simulink library "xbsIndex_r4"  (Simulink 7.1)
(part 5 of 9)

      | nport = get_param(gcbh, 'ports');
      | nin = nport(1);
      | nout = nport(2);
      | 
      |   serialized_declarations = '{''Coefficient_Binary_Point''=>''Int'',''Coefficient_Buffer_Type''=>''Int'',''Coefficient_Reload''=>''Int'',''Coefficient_Sign''=>''Int'',''Coefficient_Structure''=>''Int'',''Coefficient_Width''=>''Int'',''Coefficients''=>''DoubleVector'',''Column_Wrap_Length''=>''Int'',''Data_Buffer_Type''=>''Int'',''Display_Block_Info''=>''Int'',''Enable_Port''=>''Int'',''Filter_Type''=>''Int'',''First_Column_Length''=>''Int'',''Hardware_Oversampling''=>''Int'',''Inter_Column_Pipe_Length''=>''Int'',''Multiple_Column_Support''=>''Int'',''Number_Channels''=>''Int'',''Rate_Change''=>''Int'',''Rst_Rfd_Port''=>''Int'',''Storage''=>''Int'',''Valid_Ports''=>''Int'',''Zero_Pack_Factor''=>''Int'',''enable_debug''=>''Int'',''u_coef_cols''=>''Int'',''u_coef_rows''=>''Int'',''u_coef_sets''=>''Int'',''u_coef_type''=>''Int'',''u_latency''=>''Int'',''block_type''=>''String'',''nin''=>''Double'',''nout''=>''Double''}';
      |   xlFir_compiler_v3_0_init();
      |   ptable_ = xlblockprep(get_param(tmp_gcb, 'MaskWSVariables'));
      |   try
      |     xlBlockMoveCallback(tmp_gcbh);
      |   catch 
      |      clear global xl_updateicon_recursion_guard;
      |   end;
      | catch
      |   global dbgsysgen;
      |   if(~isempty(dbgsysgen) && dbgsysgen)
      |     e = regexprep(lasterr, '\n', '\nError: ');
      |     disp(['Error: While running MaskInit code on block ' tmp_gcb ': ' e]);
      |     error(e);
      |   end
      | end
      settings: CopyFcn=xlBlockMoveCallback(gcbh);  DeleteFcn=xlDestroyGui(gcbh);  ModelCloseFcn=xlDestroyGui(gcbh);  PreSaveFcn=xlBlockPreSaveCallback(gcbh);  PostSaveFcn=xlBlockPostSaveCallback(gcbh);  DestroyFcn=xlDestroyGui(gcbh);  OpenFcn=xlOpenGui(gcbh, 'Fir_compiler_v3_0_gui.xml', @xlremovedenablement, -1)  CloseFcn=xlDestroyGui(gcbh);  MoveFcn=xlBlockMoveCallback(gcbh);
      mask Help: eval('');xlDoc('-book','sysgen','-topic','FIR_Compiler_v3_0');
      mask StyleString: edit,edit,popup(Single_Rate|Decimation|Interpolation|Interpolated),edit,edit,edit,edit,edit,edit,popup(Signed|Unsigned),edit,edit,edit,popup(Inferred|Non_Symmetric|Symmetric|Negative_Symmetric|Half_Band),edit,checkbox,edit,checkbox,edit,checkbox,edit,checkbox,edit,checkbox,edit,checkbox,edit,popup(Automatic|Custom),edit,popup(Distributed|Block),edit,popup(Distributed|Block),edit,popup(Disabled|Custom),edit,popup(1|2|3|4|5|6|7|8|9|10|11|12|13|14|15|16),edit,edit,edit,checkbox,edit,edit,edit,edit,edit,edit,edit,edit,edit,edit,edit,edit,edit,edit,edit
      mask Display:
      | fprintf('','COMMENT: begin icon graphics');
      | patch([0 90 90 0 0 ],[0 0 134 134 0 ],[0.77 0.82 0.91 ]);
      | plot([0 90 90 0 0 ],[0 0 134 134 0 ]);
      | patch([18.3 35.64 47.64 59.64 71.64 47.64 30.3 18.3 ],[80.32 80.32 92.32 80.32 92.32 92.32 92.32 80.32 ],[1 1 1 ]);
      | patch([30.3 47.64 35.64 18.3 30.3 ],[68.32 68.32 80.32 80.32 68.32 ],[0.931 0.946 0.973 ]);
      | patch([18.3 35.64 47.64 30.3 18.3 ],[56.32 56.32 68.32 68.32 56.32 ],[1 1 1 ]);
      | patch([30.3 71.64 59.64 47.64 35.64 18.3 30.3 ],[44.32 44.32 56.32 44.32 56.32 56.32 44.32 ],[0.931 0.946 0.973 ]);
      | fprintf('','COMMENT: end icon graphics');
      | fprintf('','COMMENT: begin icon text');
      | fprintf('','COMMENT: end icon text');
  "FIR Compiler v3_1 " : S-Function  LoadFcn=xlBlockLoadCallback(gcbh);  FunctionName=sysgen  Parameters=ptable_  EnableBusSupport=off  mask(Xilinx FIR Compiler v3_1 Block){infoedit=Implements a high-speed multi-channel FIR filter.<br><br>Hardware  notes: Implemented using DSP48s hence only Virtex 4, Virtex 5 and SpartanDSP devices are supported., Filter_Type_sgadvanced=, Filter_Type=Single_Rate, Rate_Change=1, Zero_Pack_Factor=1, Number_Channels=1, Hardware_Oversampling=1, Coefficients=[1 2 3], Coefficient_Sign_sgadvanced=, Coefficient_Sign=Signed, Coefficient_Width=16, Coefficient_Binary_Point=8, Coefficient_Structure_sgadvanced=, Coefficient_Structure=Inferred, Coefficient_Reload_sgadvanced=, Coefficient_Reload=off, Display_Block_Info_sgadvanced=, Display_Block_Info=off, Valid_Ports_sgadvanced=, Valid_Ports=off, Enable_Port_sgadvanced=, Enable_Port=off, Rst_Rfd_Port_sgadvanced=, Rst_Rfd_Port=off, Output_Rounding_Mode_sgadvanced=, Output_Rounding_Mode=Full_Precision, Output_Width=48, Allow_Rounding_Approximation_sgadvanced=, Allow_Rounding_Approximation=off, dbl_ovrd_sgadvanced=, dbl_ovrd=off, Storage_sgadvanced=, Storage=Automatic, Data_Buffer_Type_sgadvanced=, Data_Buffer_Type=Distributed, Coefficient_Buffer_Type_sgadvanced=, Coefficient_Buffer_Type=Distributed, Multiple_Column_Support_sgadvanced=, Multiple_Column_Support=Disabled, Inter_Column_Pipe_Length_sgadvanced=, Inter_Column_Pipe_Length=4, First_Column_Length=32, Column_Wrap_Length=32, xl_use_area_sgadvanced=, xl_use_area=off, xl_area=[0,0,0,0,0,0,0], u_coef_rows=1, u_coef_cols=3, u_coef_sets=1, u_coef_type=1, u_latency=1, enable_debug=0, has_advanced_control=0, sggui_pos=-1,-1,-1,-1, block_type=Fir_compiler_v3_1, block_version=, sg_icon_stat=90,134,-1,-1,white,blue,0,07734,right,,[ ],[ ], sg_mask_display=|, sg_list_contents=, sg_blockgui_xml=}
      mask sg_mask_display=|
      | fprintf('','COMMENT: begin icon graphics');
      | patch([0 90 90 0 0 ],[0 0 134 134 0 ],[0.77 0.82 0.91 ]);
      | plot([0 90 90 0 0 ],[0 0 134 134 0 ]);
      | patch([18.3 35.64 47.64 59.64 71.64 47.64 30.3 18.3 ],[80.32 80.32 92.32 80.32 92.32 92.32 92.32 80.32 ],[1 1 1 ]);
      | patch([30.3 47.64 35.64 18.3 30.3 ],[68.32 68.32 80.32 80.32 68.32 ],[0.931 0.946 0.973 ]);
      | patch([18.3 35.64 47.64 30.3 18.3 ],[56.32 56.32 68.32 68.32 56.32 ],[1 1 1 ]);
      | patch([30.3 71.64 59.64 47.64 35.64 18.3 30.3 ],[44.32 44.32 56.32 44.32 56.32 56.32 44.32 ],[0.931 0.946 0.973 ]);
      | fprintf('','COMMENT: end icon graphics');
      | fprintf('','COMMENT: begin icon text');
      | fprintf('','COMMENT: end icon text');
      mask prompts: infoedit ""; Filter_Type_sgadvanced ""; Filter_Type "Filter type"; Rate_Change "Sample rate change"; Zero_Pack_Factor "Zero Packing Factor"; Number_Channels "Number of channels"; Hardware_Oversampling "Hardware over-sampling rate"; Coefficients "Coefficient vector"; Coefficient_Sign_sgadvanced ""; Coefficient_Sign "Arithmetic type"; Coefficient_Width "Number of bits"; Coefficient_Binary_Point "Binary point"; Coefficient_Structure_sgadvanced ""; Coefficient_Structure "Structure"; Coefficient_Reload_sgadvanced ""; Coefficient_Reload "Use reloadable coefficients"; Display_Block_Info_sgadvanced ""; Display_Block_Info "Display filter information on block icon"; Valid_Ports_sgadvanced ""; Valid_Ports "Provide valid ports"; Enable_Port_sgadvanced ""; Enable_Port "Provide <tt>en</tt> port"; Rst_Rfd_Port_sgadvanced ""; Rst_Rfd_Port "Provide <tt>rst</tt> port"; Output_Rounding_Mode_sgadvanced ""; Output_Rounding_Mode "Rounding mode"; Output_Width "Output width"; Allow_Rounding_Approximation_sgadvanced ""; Allow_Rounding_Approximation "Allow rounding approximation"; dbl_ovrd_sgadvanced ""; dbl_ovrd "Override with doubles"; Storage_sgadvanced ""; Storage ""; Data_Buffer_Type_sgadvanced ""; Data_Buffer_Type "Data buffer"; Coefficient_Buffer_Type_sgadvanced ""; Coefficient_Buffer_Type "Coefficient buffer"; Multiple_Column_Support_sgadvanced ""; Multiple_Column_Support ""; Inter_Column_Pipe_Length_sgadvanced ""; Inter_Column_Pipe_Length "Cross column pipelining"; First_Column_Length "First column length"; Column_Wrap_Length "Column wrap length"; xl_use_area_sgadvanced ""; xl_use_area "Define FPGA area for resource estimation"; xl_area "FPGA area [slices, FFs, BRAMs, LUTs, IOBs, emb. mults, TBUFs]"; u_coef_rows ""; u_coef_cols ""; u_coef_sets ""; u_coef_type ""; u_latency ""; enable_debug ""; has_advanced_control ""; sggui_pos ""; block_type ""; block_version ""; sg_icon_stat ""; sg_mask_display ""; sg_list_contents ""; sg_blockgui_xml ""
      mask help:
      | Implements a high-speed multi-channel FIR filter.
      |
      | Hardware  notes: Implemented using DSP48s hence only Virtex 4, Virtex 5 and SpartanDSP devices are supported.
      mask init:
      | try
      |   tmp_gcb = gcb;
      |   tmp_gcbh = gcbh;
      |   if (strcmp('SysGenIndex',get_param(bdroot(tmp_gcbh),'tag')) && ~isempty(regexp(bdroot(tmp_gcb), '^xbs', 'once')))
      |     return;
      |   end;
      |   xlMungeMaskParams;
      |   block_config = 'sysgen_blockset:Removed_config';
      | 
      |   block_type='Fir_compiler_v3_1';
      | nport = get_param(gcbh, 'ports');
      | nin = nport(1);
      | nout = nport(2);
      | 
      |   serialized_declarations = '{''Allow_Rounding_Approximation''=>''Int'',''Coefficient_Binary_Point''=>''Int'',''Coefficient_Buffer_Type''=>''Int'',''Coefficient_Reload''=>''Int'',''Coefficient_Sign''=>''Int'',''Coefficient_Structure''=>''Int'',''Coefficient_Width''=>''Int'',''Coefficients''=>''DoubleVector'',''Column_Wrap_Length''=>''Int'',''Data_Buffer_Type''=>''Int'',''Display_Block_Info''=>''Int'',''Enable_Port''=>''Int'',''Filter_Type''=>''Int'',''First_Column_Length''=>''Int'',''Hardware_Oversampling''=>''Int'',''Inter_Column_Pipe_Length''=>''Int'',''Multiple_Column_Support''=>''Int'',''Number_Channels''=>''Int'',''Output_Rounding_Mode''=>''Int'',''Output_Width''=>''Int'',''Rate_Change''=>''Int'',''Rst_Rfd_Port''=>''Int'',''Storage''=>''Int'',''Valid_Ports''=>''Int'',''Zero_Pack_Factor''=>''Int'',''enable_debug''=>''Int'',''u_coef_cols''=>''Int'',''u_coef_rows''=>''Int'',''u_coef_sets''=>''Int'',''u_coef_type''=>''Int'',''u_latency''=>''Int'',''block_type''=>''String'',''nin''=>''Double'',''nout''=>''Double''}';
      |   xlFir_compiler_v3_0_init();
      |   ptable_ = xlblockprep(get_param(tmp_gcb, 'MaskWSVariables'));
      |   try
      |     xlBlockMoveCallback(tmp_gcbh);
      |   catch 
      |      clear global xl_updateicon_recursion_guard;
      |   end;
      | catch
      |   global dbgsysgen;
      |   if(~isempty(dbgsysgen) && dbgsysgen)
      |     e = regexprep(lasterr, '\n', '\nError: ');
      |     disp(['Error: While running MaskInit code on block ' tmp_gcb ': ' e]);
      |     error(e);
      |   end
      | end
      settings: CopyFcn=xlBlockMoveCallback(gcbh);  DeleteFcn=xlDestroyGui(gcbh);  ModelCloseFcn=xlDestroyGui(gcbh);  PreSaveFcn=xlBlockPreSaveCallback(gcbh);  PostSaveFcn=xlBlockPostSaveCallback(gcbh);  DestroyFcn=xlDestroyGui(gcbh);  OpenFcn=xlOpenGui(gcbh, 'Fir_compiler_v3_1_gui.xml', @xlremovedenablement, -1)  CloseFcn=xlDestroyGui(gcbh);  MoveFcn=xlBlockMoveCallback(gcbh);
      mask Help: eval('');xlDoc('-book','sysgen','-topic','FIR_Compiler_v3_1');
      mask StyleString: edit,edit,popup(Single_Rate|Decimation|Interpolation|Interpolated),edit,edit,edit,edit,edit,edit,popup(Signed|Unsigned),edit,edit,edit,popup(Inferred|Non_Symmetric|Symmetric|Negative_Symmetric|Half_Band),edit,checkbox,edit,checkbox,edit,checkbox,edit,checkbox,edit,checkbox,edit,popup(Full_Precision|Truncated_LSBs|Symmetric_Rounding_to_Zero|Symmetric_Rounding_to_Infinity|Convergent_Rounding_to_Even|Convergent_Rounding_to_Odd|Non_Symmetric_Rounding_Down|Non_Symmetric_Rounding_Up),edit,edit,checkbox,edit,checkbox,edit,popup(Automatic|Custom),edit,popup(Distributed|Block),edit,popup(Distributed|Block),edit,popup(Disabled|Custom),edit,popup(1|2|3|4|5|6|7|8|9|10|11|12|13|14|15|16),edit,edit,edit,checkbox,edit,edit,edit,edit,edit,edit,edit,edit,edit,edit,edit,edit,edit,edit,edit
      mask Display:
      | fprintf('','COMMENT: begin icon graphics');
      | patch([0 90 90 0 0 ],[0 0 134 134 0 ],[0.77 0.82 0.91 ]);
      | plot([0 90 90 0 0 ],[0 0 134 134 0 ]);
      | patch([18.3 35.64 47.64 59.64 71.64 47.64 30.3 18.3 ],[80.32 80.32 92.32 80.32 92.32 92.32 92.32 80.32 ],[1 1 1 ]);
      | patch([30.3 47.64 35.64 18.3 30.3 ],[68.32 68.32 80.32 80.32 68.32 ],[0.931 0.946 0.973 ]);
      | patch([18.3 35.64 47.64 30.3 18.3 ],[56.32 56.32 68.32 68.32 56.32 ],[1 1 1 ]);
      | patch([30.3 71.64 59.64 47.64 35.64 18.3 30.3 ],[44.32 44.32 56.32 44.32 56.32 56.32 44.32 ],[0.931 0.946 0.973 ]);
      | fprintf('','COMMENT: end icon graphics');
      | fprintf('','COMMENT: begin icon text');
      | fprintf('','COMMENT: end icon text');
  "FIR Compiler v3_2 " : S-Function  LoadFcn=xlBlockLoadCallback(gcbh);  FunctionName=sysgen  Parameters=ptable_  EnableBusSupport=off  mask(Xilinx FIR Compiler v3_2 Block){infoedit=Implements a high-speed multi-channel FIR filter.<br><br>Hardware  notes: Implemented using DSP48s hence only Virtex 4, Virtex 5 and SpartanDSP devices are supported., Filter_Type_sgadvanced=, Filter_Type=Single_Rate, Rate_Change=1, Zero_Pack_Factor=1, Number_Channels=1, Hardware_Oversampling=1, Coefficients=[1 2 3], Coefficient_Sign_sgadvanced=, Coefficient_Sign=Signed, Coefficient_Width=16, Coefficient_Binary_Point=8, Coefficient_Structure_sgadvanced=, Coefficient_Structure=Inferred, Coefficient_Reload_sgadvanced=, Coefficient_Reload=off, Display_Block_Info_sgadvanced=, Display_Block_Info=off, Valid_Ports_sgadvanced=, Valid_Ports=off, Enable_Port_sgadvanced=, Enable_Port=off, Rst_Rfd_Port_sgadvanced=, Rst_Rfd_Port=off, Output_Rounding_Mode_sgadvanced=, Output_Rounding_Mode=Full_Precision, Output_Width=48, Allow_Rounding_Approximation_sgadvanced=, Allow_Rounding_Approximation=off, dbl_ovrd_sgadvanced=, dbl_ovrd=off, Storage_sgadvanced=, Storage=Automatic, Data_Buffer_Type_sgadvanced=, Data_Buffer_Type=Distributed, Coefficient_Buffer_Type_sgadvanced=, Coefficient_Buffer_Type=Distributed, Multiple_Column_Support_sgadvanced=, Multiple_Column_Support=Disabled, Inter_Column_Pipe_Length_sgadvanced=, Inter_Column_Pipe_Length=4, First_Column_Length=32, Column_Wrap_Length=32, xl_use_area_sgadvanced=, xl_use_area=off, xl_area=[0,0,0,0,0,0,0], u_coef_rows=1, u_coef_cols=3, u_coef_sets=1, u_coef_type=1, u_latency=1, enable_debug=0, has_advanced_control=0, sggui_pos=-1,-1,-1,-1, block_type=Fir_compiler_v3_2, block_version=, sg_icon_stat=90,134,-1,-1,white,blue,0,07734,right,,[ ],[ ], sg_mask_display=|, sg_list_contents=, sg_blockgui_xml=}
      mask sg_mask_display=|
      | fprintf('','COMMENT: begin icon graphics');
      | patch([0 90 90 0 0 ],[0 0 134 134 0 ],[0.77 0.82 0.91 ]);
      | plot([0 90 90 0 0 ],[0 0 134 134 0 ]);
      | patch([18.3 35.64 47.64 59.64 71.64 47.64 30.3 18.3 ],[80.32 80.32 92.32 80.32 92.32 92.32 92.32 80.32 ],[1 1 1 ]);
      | patch([30.3 47.64 35.64 18.3 30.3 ],[68.32 68.32 80.32 80.32 68.32 ],[0.931 0.946 0.973 ]);
      | patch([18.3 35.64 47.64 30.3 18.3 ],[56.32 56.32 68.32 68.32 56.32 ],[1 1 1 ]);
      | patch([30.3 71.64 59.64 47.64 35.64 18.3 30.3 ],[44.32 44.32 56.32 44.32 56.32 56.32 44.32 ],[0.931 0.946 0.973 ]);
      | fprintf('','COMMENT: end icon graphics');
      | fprintf('','COMMENT: begin icon text');
      | fprintf('','COMMENT: end icon text');
      mask prompts: infoedit ""; Filter_Type_sgadvanced ""; Filter_Type "Filter type"; Rate_Change "Sample rate change"; Zero_Pack_Factor "Zero Packing Factor"; Number_Channels "Number of channels"; Hardware_Oversampling "Hardware over-sampling rate"; Coefficients "Coefficient vector"; Coefficient_Sign_sgadvanced ""; Coefficient_Sign "Arithmetic type"; Coefficient_Width "Number of bits"; Coefficient_Binary_Point "Binary point"; Coefficient_Structure_sgadvanced ""; Coefficient_Structure "Structure"; Coefficient_Reload_sgadvanced ""; Coefficient_Reload "Use reloadable coefficients"; Display_Block_Info_sgadvanced ""; Display_Block_Info "Display filter information on block icon"; Valid_Ports_sgadvanced ""; Valid_Ports "Provide valid ports"; Enable_Port_sgadvanced ""; Enable_Port "Provide <tt>en</tt> port"; Rst_Rfd_Port_sgadvanced ""; Rst_Rfd_Port "Provide <tt>rst</tt> port"; Output_Rounding_Mode_sgadvanced ""; Output_Rounding_Mode "Rounding mode"; Output_Width "Output width"; Allow_Rounding_Approximation_sgadvanced ""; Allow_Rounding_Approximation "Allow rounding approximation"; dbl_ovrd_sgadvanced ""; dbl_ovrd "Override with doubles"; Storage_sgadvanced ""; Storage ""; Data_Buffer_Type_sgadvanced ""; Data_Buffer_Type "Data buffer"; Coefficient_Buffer_Type_sgadvanced ""; Coefficient_Buffer_Type "Coefficient buffer"; Multiple_Column_Support_sgadvanced ""; Multiple_Column_Support ""; Inter_Column_Pipe_Length_sgadvanced ""; Inter_Column_Pipe_Length "Cross column pipelining"; First_Column_Length "First column length"; Column_Wrap_Length "Column wrap length"; xl_use_area_sgadvanced ""; xl_use_area "Define FPGA area for resource estimation"; xl_area "FPGA area [slices, FFs, BRAMs, LUTs, IOBs, emb. mults, TBUFs]"; u_coef_rows ""; u_coef_cols ""; u_coef_sets ""; u_coef_type ""; u_latency ""; enable_debug ""; has_advanced_control ""; sggui_pos ""; block_type ""; block_version ""; sg_icon_stat ""; sg_mask_display ""; sg_list_contents ""; sg_blockgui_xml ""
      mask help:
      | Implements a high-speed multi-channel FIR filter.
      |
      | Hardware  notes: Implemented using DSP48s hence only Virtex 4, Virtex 5 and SpartanDSP devices are supported.
      mask init:
      | try
      |   tmp_gcb = gcb;
      |   tmp_gcbh = gcbh;
      |   if (strcmp('SysGenIndex',get_param(bdroot(tmp_gcbh),'tag')) && ~isempty(regexp(bdroot(tmp_gcb), '^xbs', 'once')))
      |     return;
      |   end;
      |   xlMungeMaskParams;
      |   block_config = 'sysgen_blockset:Removed_config';
      | 
      |   block_type='Fir_compiler_v3_2';
      | nport = get_param(gcbh, 'ports');
      | nin = nport(1);
      | nout = nport(2);
      | 
      |   serialized_declarations = '{''Allow_Rounding_Approximation''=>''Int'',''Coefficient_Binary_Point''=>''Int'',''Coefficient_Buffer_Type''=>''Int'',''Coefficient_Reload''=>''Int'',''Coefficient_Sign''=>''Int'',''Coefficient_Structure''=>''Int'',''Coefficient_Width''=>''Int'',''Coefficients''=>''DoubleVector'',''Column_Wrap_Length''=>''Int'',''Data_Buffer_Type''=>''Int'',''Display_Block_Info''=>''Int'',''Enable_Port''=>''Int'',''Filter_Type''=>''Int'',''First_Column_Length''=>''Int'',''Hardware_Oversampling''=>''Int'',''Inter_Column_Pipe_Length''=>''Int'',''Multiple_Column_Support''=>''Int'',''Number_Channels''=>''Int'',''Output_Rounding_Mode''=>''Int'',''Output_Width''=>''Int'',''Rate_Change''=>''Int'',''Rst_Rfd_Port''=>''Int'',''Storage''=>''Int'',''Valid_Ports''=>''Int'',''Zero_Pack_Factor''=>''Int'',''enable_debug''=>''Int'',''u_coef_cols''=>''Int'',''u_coef_rows''=>''Int'',''u_coef_sets''=>''Int'',''u_coef_type''=>''Int'',''u_latency''=>''Int'',''block_type''=>''String'',''nin''=>''Double'',''nout''=>''Double''}';
      |   xlFir_compiler_v3_0_init();
      |   ptable_ = xlblockprep(get_param(tmp_gcb, 'MaskWSVariables'));
      |   try
      |     xlBlockMoveCallback(tmp_gcbh);
      |   catch 
      |      clear global xl_updateicon_recursion_guard;
      |   end;
      | catch
      |   global dbgsysgen;
      |   if(~isempty(dbgsysgen) && dbgsysgen)
      |     e = regexprep(lasterr, '\n', '\nError: ');
      |     disp(['Error: While running MaskInit code on block ' tmp_gcb ': ' e]);
      |     error(e);
      |   end
      | end
      settings: CopyFcn=xlBlockMoveCallback(gcbh);  DeleteFcn=xlDestroyGui(gcbh);  ModelCloseFcn=xlDestroyGui(gcbh);  PreSaveFcn=xlBlockPreSaveCallback(gcbh);  PostSaveFcn=xlBlockPostSaveCallback(gcbh);  DestroyFcn=xlDestroyGui(gcbh);  OpenFcn=xlOpenGui(gcbh, 'Fir_compiler_v3_2_gui.xml', @xlremovedenablement, -1)  CloseFcn=xlDestroyGui(gcbh);  MoveFcn=xlBlockMoveCallback(gcbh);
      mask Help: eval('');xlDoc('-book','sysgen','-topic','FIR_Compiler_v3_2');
      mask StyleString: edit,edit,popup(Single_Rate|Decimation|Interpolation|Interpolated),edit,edit,edit,edit,edit,edit,popup(Signed|Unsigned),edit,edit,edit,popup(Inferred|Non_Symmetric|Symmetric|Negative_Symmetric|Half_Band),edit,checkbox,edit,checkbox,edit,checkbox,edit,checkbox,edit,checkbox,edit,popup(Full_Precision|Truncated_LSBs|Symmetric_Rounding_to_Zero|Symmetric_Rounding_to_Infinity|Convergent_Rounding_to_Even|Convergent_Rounding_to_Odd|Non_Symmetric_Rounding_Down|Non_Symmetric_Rounding_Up),edit,edit,checkbox,edit,checkbox,edit,popup(Automatic|Custom),edit,popup(Distributed|Block),edit,popup(Distributed|Block),edit,popup(Disabled|Custom),edit,popup(1|2|3|4|5|6|7|8|9|10|11|12|13|14|15|16),edit,edit,edit,checkbox,edit,edit,edit,edit,edit,edit,edit,edit,edit,edit,edit,edit,edit,edit,edit
      mask Display:
      | fprintf('','COMMENT: begin icon graphics');
      | patch([0 90 90 0 0 ],[0 0 134 134 0 ],[0.77 0.82 0.91 ]);
      | plot([0 90 90 0 0 ],[0 0 134 134 0 ]);
      | patch([18.3 35.64 47.64 59.64 71.64 47.64 30.3 18.3 ],[80.32 80.32 92.32 80.32 92.32 92.32 92.32 80.32 ],[1 1 1 ]);
      | patch([30.3 47.64 35.64 18.3 30.3 ],[68.32 68.32 80.32 80.32 68.32 ],[0.931 0.946 0.973 ]);
      | patch([18.3 35.64 47.64 30.3 18.3 ],[56.32 56.32 68.32 68.32 56.32 ],[1 1 1 ]);
      | patch([30.3 71.64 59.64 47.64 35.64 18.3 30.3 ],[44.32 44.32 56.32 44.32 56.32 56.32 44.32 ],[0.931 0.946 0.973 ]);
      | fprintf('','COMMENT: end icon graphics');
      | fprintf('','COMMENT: begin icon text');
      | fprintf('','COMMENT: end icon text');
  "Fast Fourier Transform 6.0 " : S-Function  LoadFcn=xlBlockLoadCallback(gcbh);  FunctionName=sysgen  Parameters=ptable_  EnableBusSupport=off  mask(Xilinx Fast Fourier Transform 6.0 Block){transform_length=1024, implementation_options=pipelined_streaming_io, run_time_configurable_transform_length=off, phase_factor_width=16, scaling_options=scaled, rounding_modes=truncation, output_ordering=bit_reversed_order, cyclic_prefix_insertion=off, en=off, rst=off, ovflo=off, memory_options_data=block_ram, memory_options_phase_factors=block_ram, number_of_stages_using_block_ram_for_data_and_phase_factors=1, memory_options_reorder=block_ram, memory_options_hybrid=off, optimize_for_speed_using_xtreme_dsp_slices=off, fast_complex_mult=off, fast_butterfly=off, xl_use_area=off, xl_area=[0,0,0,0,0,0,0], target_clock_frequency=250, simulation_type=external_xfix, simulation_model=fftv6_CModel:fftv6_cmodel, ip_name=Fast Fourier Transform, ip_version=6.0, dsptool_ready=true, input_ordering=natural_order, ce=true, sclr=0, wrapper_available=true, port_translation_map={ 'ce' => 'en', 'sclr' => 'rst' }, ipcore_fpga_part=xlipgetpartsetting(gcb, {'virtex4', 'xc4vsx35', '-10', 'ff668'}), target_data_throughput=50, channels=1, input_width=16, has_advanced_control=0, sggui_pos=-1,-1,-1,-1, block_type=xfft_v6_0, block_version=, sg_icon_stat=95,142,-1,-1,white,blue,0,07734,right,,[ ],[ ], sg_mask_display=|, sg_list_contents=, sg_blockgui_xml=}
      mask sg_mask_display=|
      | fprintf('','COMMENT: begin icon graphics');
      | patch([0 95 95 0 0 ],[0 0 142 142 0 ],[0.77 0.82 0.91 ]);
      | plot([0 95 95 0 0 ],[0 0 142 142 0 ]);
      | patch([18.075 36.86 49.86 62.86 75.86 49.86 31.075 18.075 ],[85.43 85.43 98.43 85.43 98.43 98.43 98.43 85.43 ],[1 1 1 ]);
      | patch([31.075 49.86 36.86 18.075 31.075 ],[72.43 72.43 85.43 85.43 72.43 ],[0.931 0.946 0.973 ]);
      | patch([18.075 36.86 49.86 31.075 18.075 ],[59.43 59.43 72.43 72.43 59.43 ],[1 1 1 ]);
      | patch([31.075 75.86 62.86 49.86 36.86 18.075 31.075 ],[46.43 46.43 59.43 46.43 59.43 59.43 46.43 ],[0.931 0.946 0.973 ]);
      | fprintf('','COMMENT: end icon graphics');
      | fprintf('','COMMENT: begin icon text');
      | fprintf('','COMMENT: end icon text');
      mask prompts: transform_length "Transform length"; implementation_options "Implementation options"; run_time_configurable_transform_length "Run time configurable transform length"; phase_factor_width "Phase factor width"; scaling_options "Scaling options"; rounding_modes "Rounding modes"; output_ordering "Output ordering"; cyclic_prefix_insertion "Cyclic prefix insertion"; memory_options_data "Data"; memory_options_phase_factors "Phase factors"; number_of_stages_using_block_ram_for_data_and_phase_factors "Number of stages using Block RAM"; memory_options_reorder "Reorder buffer"; memory_options_hybrid "Optimize Block RAM count using hybrid memories"; optimize_for_speed_using_xtreme_dsp_slices "Optimize for speed using xtreme dsp slices"; fast_complex_mult "Complex multiplication"; fast_butterfly "Butterfly arithmetic"; xl_use_area "Define FPGA area for resource estimation"; xl_area "FPGA area [slices, FFs, BRAMs, LUTs, IOBs, emb. mults, TBUFs]"; target_clock_frequency ""; simulation_type ""; simulation_model ""; ip_name ""; ip_version ""; dsptool_ready ""; input_ordering ""; ce ""; sclr ""; wrapper_available ""; port_translation_map ""; ipcore_fpga_part ""; target_data_throughput ""; channels ""; input_width ""; has_advanced_control ""; sggui_pos ""; block_type ""; block_version ""; sg_icon_stat ""; sg_mask_display ""; sg_list_contents ""; sg_blockgui_xml ""
      mask help: Xilinx Fast Fourier Transform 6.0
      mask init:
      | try
      |   tmp_gcb = gcb;
      |   tmp_gcbh = gcbh;
      |   if (strcmp('SysGenIndex',get_param(bdroot(tmp_gcbh),'tag')) && ~isempty(regexp(bdroot(tmp_gcb), '^xbs', 'once')))
      |     return;
      |   end;
      |   xlMungeMaskParams;
      |   block_config = 'sysgen_blockset:Removed_config';
      | 
      |   block_type='xfft_v6_0';
      | nport = get_param(gcbh, 'ports');
      | nin = nport(1);
      | nout = nport(2);
      | 
      |   serialized_declarations = '{''ce''=>''Bool'',''channels''=>''String'',''cyclic_prefix_insertion''=>''Bool'',''dsptool_ready''=>''Bool'',''en''=>''Bool'',''fast_butterfly''=>''Bool'',''fast_complex_mult''=>''Bool'',''implementation_options''=>''String'',''input_ordering''=>''String'',''input_width''=>''String'',''ip_name''=>''String'',''ip_version''=>''String'',''ipcore_fpga_part''=>''StringVector'',''memory_options_data''=>''String'',''memory_options_hybrid''=>''Bool'',''memory_options_phase_factors''=>''String'',''memory_options_reorder''=>''String'',''number_of_stages_using_block_ram_for_data_and_phase_factors''=>''String'',''optimize_for_speed_using_xtreme_dsp_slices''=>''Bool'',''output_ordering''=>''String'',''ovflo''=>''Bool'',''phase_factor_width''=>''String'',''port_translation_map''=>''String'',''rounding_modes''=>''String'',''rst''=>''Bool'',''run_time_configurable_transform_length''=>''Bool'',''scaling_options''=>''String'',''sclr''=>''Bool'',''simulation_model''=>''String'',''simulation_type''=>''String'',''target_clock_frequency''=>''Int'',''target_data_throughput''=>''Int'',''transform_length''=>''String'',''wrapper_available''=>''Bool'',''xl_use_area''=>''Bool'',''block_type''=>''String'',''nin''=>''Double'',''nout''=>''Double''}';
      |   xlfft_v6_0_init();
      |   ptable_ = xlblockprep(get_param(tmp_gcb, 'MaskWSVariables'));
      |   try
      |     xlBlockMoveCallback(tmp_gcbh);
      |   catch 
      |      clear global xl_updateicon_recursion_guard;
      |   end;
      | catch
      |   global dbgsysgen;
      |   if(~isempty(dbgsysgen) && dbgsysgen)
      |     e = regexprep(lasterr, '\n', '\nError: ');
      |     disp(['Error: While running MaskInit code on block ' tmp_gcb ': ' e]);
      |     error(e);
      |   end
      | end
      settings: CopyFcn=xlBlockMoveCallback(gcbh);  DeleteFcn=xlDestroyGui(gcbh);  ModelCloseFcn=xlDestroyGui(gcbh);  PreSaveFcn=xlBlockPreSaveCallback(gcbh);  PostSaveFcn=xlBlockPostSaveCallback(gcbh);  DestroyFcn=xlDestroyGui(gcbh);  OpenFcn=xlOpenGui(gcbh, 'fft_v6_0_gui.xml', @xlremovedenablement, -1)  CloseFcn=xlDestroyGui(gcbh);  MoveFcn=xlBlockMoveCallback(gcbh);
      mask Help: eval('');xlDoc('-book','sysgen','-topic','Fast_Fourier_Transform_6_0');
      mask StyleString: popup(8|16|32|64|128|256|512|1024|2048|4096|8192|16384|32768|65536),popup(pipelined_streaming_io|radix_4_burst_io|radix_2_burst_io|radix_2_lite_burst_io),checkbox,popup(8|9|10|11|12|13|14|15|16|17|18|19|20|21|22|23|24|25|26|27|28|29|30|31|32|33|34),popup(unscaled|scaled|block_floating_point),popup(truncation|convergent_rounding),popup(bit_reversed_order|natural_order),checkbox,checkbox,checkbox,checkbox,popup(block_ram|distributed_ram),popup(block_ram|distributed_ram),popup(0|1|2|3|4|5|6|7|8|9|10|11),popup(block_ram|distributed_ram),checkbox,checkbox,checkbox,checkbox,checkbox,edit,edit,edit,edit,edit,edit,edit,edit,edit,edit,edit,edit,edit,edit,edit,edit,edit,edit,edit,edit,edit,edit,edit,edit
      mask Display:
      | fprintf('','COMMENT: begin icon graphics');
      | patch([0 95 95 0 0 ],[0 0 142 142 0 ],[0.77 0.82 0.91 ]);
      | plot([0 95 95 0 0 ],[0 0 142 142 0 ]);
      | patch([18.075 36.86 49.86 62.86 75.86 49.86 31.075 18.075 ],[85.43 85.43 98.43 85.43 98.43 98.43 98.43 85.43 ],[1 1 1 ]);
      | patch([31.075 49.86 36.86 18.075 31.075 ],[72.43 72.43 85.43 85.43 72.43 ],[0.931 0.946 0.973 ]);
      | patch([18.075 36.86 49.86 31.075 18.075 ],[59.43 59.43 72.43 72.43 59.43 ],[1 1 1 ]);
      | patch([31.075 75.86 62.86 49.86 36.86 18.075 31.075 ],[46.43 46.43 59.43 46.43 59.43 59.43 46.43 ],[0.931 0.946 0.973 ]);
      | fprintf('','COMMENT: end icon graphics');
      | fprintf('','COMMENT: begin icon text');
      | fprintf('','COMMENT: end icon text');
  "Fast Fourier Transform 7.0 " : S-Function  LoadFcn=xlBlockLoadCallback(gcbh);  FunctionName=sysgen  Parameters=ptable_  EnableBusSupport=off  mask(Xilinx Fast Fourier Transform 7.0 Block){transform_length=1024, implementation_options=pipelined_streaming_io, target_clock_frequency=250, target_data_throughput=50, run_time_configurable_transform_length=off, phase_factor_width=16, scaling_options=scaled, rounding_modes=truncation, output_ordering=bit_reversed_order, cyclic_prefix_insertion=off, ce=off, sclr=off, ovflo=off, input_data_offset=no_offset, memory_options_data=block_ram, memory_options_phase_factors=block_ram, number_of_stages_using_block_ram_for_data_and_phase_factors=1, memory_options_reorder=block_ram, memory_options_hybrid=off, complex_mult_type=use_mults_resources, butterfly_type=use_luts, xl_use_area=off, xl_area=[0,0,0,0,0,0,0], channels=1, input_ordering=natural_order, input_width=16, simulation_type=external_xfix, simulation_model=fftv7_CModel:fftv7_cmodel, ip_name=Fast Fourier Transform, ip_version=7.0, dsptool_ready=true, wrapper_available=true, port_translation_map={ 'ce' => 'en', 'sclr' => 'rst' }, ipcore_fpga_part=xlipgetpartsetting(gcb, {'virtex4', 'xc4vsx35', '-10', 'ff668'}), has_advanced_control=0, sggui_pos=-1,-1,-1,-1, block_type=xfft_v7_0, block_version=, sg_icon_stat=95,142,7,9,white,blue,0,c08fcb17,right,,[ ],[ ], sg_mask_display=|, sg_list_contents=, sg_blockgui_xml=}
      mask sg_mask_display=|
      | fprintf('','COMMENT: begin icon graphics');
      | patch([0 95 95 0 0 ],[0 0 142 142 0 ],[0.77 0.82 0.91 ]);
      | plot([0 95 95 0 0 ],[0 0 142 142 0 ]);
      | patch([18.075 36.86 49.86 62.86 75.86 49.86 31.075 18.075 ],[85.43 85.43 98.43 85.43 98.43 98.43 98.43 85.43 ],[1 1 1 ]);
      | patch([31.075 49.86 36.86 18.075 31.075 ],[72.43 72.43 85.43 85.43 72.43 ],[0.931 0.946 0.973 ]);
      | patch([18.075 36.86 49.86 31.075 18.075 ],[59.43 59.43 72.43 72.43 59.43 ],[1 1 1 ]);
      | patch([31.075 75.86 62.86 49.86 36.86 18.075 31.075 ],[46.43 46.43 59.43 46.43 59.43 59.43 46.43 ],[0.931 0.946 0.973 ]);
      | fprintf('','COMMENT: end icon graphics');
      | fprintf('','COMMENT: begin icon text');
      | color('black');port_label('input',1,'xn_re');
      | color('black');port_label('input',2,'xn_im');
      | color('black');port_label('input',3,'start');
      | color('black');port_label('input',4,'fwd_inv');
      | color('black');port_label('input',5,'fwd_inv_we');
      | color('black');port_label('input',6,'scale_sch');
      | color('black');port_label('input',7,'scale_sch_we');
      | color('black');port_label('output',1,'xk_re');
      | color('black');port_label('output',2,'xk_im');
      | color('black');port_label('output',3,'xn_index');
      | color('black');port_label('output',4,'xk_index');
      | color('black');port_label('output',5,'rfd');
      | color('black');port_label('output',6,'busy');
      | color('black');port_label('output',7,'dv');
      | color('black');port_label('output',8,'edone');
      | color('black');port_label('output',9,'done');
      | fprintf('','COMMENT: end icon text');
      mask prompts: transform_length ""; implementation_options ""; target_clock_frequency "Target clock frequency(MHz)"; target_data_throughput "Target data throughput(MSPS)"; run_time_configurable_transform_length "Run Time Configurable Transform Length"; phase_factor_width "Phase Factor Width"; scaling_options ""; rounding_modes ""; output_ordering ""; cyclic_prefix_insertion "Cyclic Prefix Insertion"; ce "en"; sclr "rst"; input_data_offset ""; memory_options_data ""; memory_options_phase_factors ""; number_of_stages_using_block_ram_for_data_and_phase_factors ""; memory_options_reorder ""; memory_options_hybrid "Optimize Block RAM count using hybrid memories"; complex_mult_type ""; butterfly_type ""; xl_use_area "Define FPGA area for resource estimation"; xl_area "FPGA area [slices, FFs, BRAMs, LUTs, IOBs, emb. mults, TBUFs]"; channels ""; input_ordering ""; input_width ""; simulation_type ""; simulation_model ""; ip_name ""; ip_version ""; dsptool_ready ""; wrapper_available ""; port_translation_map ""; ipcore_fpga_part ""; has_advanced_control ""; sggui_pos ""; block_type ""; block_version ""; sg_icon_stat ""; sg_mask_display ""; sg_list_contents ""; sg_blockgui_xml ""
      mask help: Xilinx Fast Fourier Transform 7.0
      mask init:
      | try
      |   tmp_gcb = gcb;
      |   tmp_gcbh = gcbh;
      |   if (strcmp('SysGenIndex',get_param(bdroot(tmp_gcbh),'tag')) && ~isempty(regexp(bdroot(tmp_gcb), '^xbs', 'once')))
      |     return;
      |   end;
      |   xlMungeMaskParams;
      |   block_config = 'sysgen:coregenimport_config';
      | 
      |   block_type='xfft_v7_0';
      | 
      |   serialized_declarations = '{''butterfly_type''=>''String'',''ce''=>''Bool'',''channels''=>''String'',''complex_mult_type''=>''String'',''cyclic_prefix_insertion''=>''Bool'',''dsptool_ready''=>''Bool'',''implementation_options''=>''String'',''input_data_offset''=>''String'',''input_ordering''=>''String'',''input_width''=>''String'',''ip_name''=>''String'',''ip_version''=>''String'',''ipcore_fpga_part''=>''StringVector'',''memory_options_data''=>''String'',''memory_options_hybrid''=>''Bool'',''memory_options_phase_factors''=>''String'',''memory_options_reorder''=>''String'',''number_of_stages_using_block_ram_for_data_and_phase_factors''=>''String'',''output_ordering''=>''String'',''ovflo''=>''Bool'',''phase_factor_width''=>''String'',''port_translation_map''=>''String'',''rounding_modes''=>''String'',''run_time_configurable_transform_length''=>''Bool'',''scaling_options''=>''String'',''sclr''=>''Bool'',''simulation_model''=>''String'',''simulation_type''=>''String'',''target_clock_frequency''=>''Int'',''target_data_throughput''=>''Int'',''transform_length''=>''String'',''wrapper_available''=>''Bool'',''xl_use_area''=>''Bool'',''block_type''=>''String''}';
      |   ptable_ = xlblockprep(get_param(tmp_gcb, 'MaskWSVariables'));
      |   try
      |     xlBlockMoveCallback(tmp_gcbh);
      |   catch 
      |      clear global xl_updateicon_recursion_guard;
      |   end;
      | catch
      |   global dbgsysgen;
      |   if(~isempty(dbgsysgen) && dbgsysgen)
      |     e = regexprep(lasterr, '\n', '\nError: ');
      |     disp(['Error: While running MaskInit code on block ' tmp_gcb ': ' e]);
      |     error(e);
      |   end
      | end
      settings: CopyFcn=xlBlockMoveCallback(gcbh);  DeleteFcn=xlDestroyGui(gcbh);  ModelCloseFcn=xlDestroyGui(gcbh);  PreSaveFcn=xlBlockPreSaveCallback(gcbh);  PostSaveFcn=xlBlockPostSaveCallback(gcbh);  DestroyFcn=xlDestroyGui(gcbh);  OpenFcn=xlOpenGui(gcbh, 'fft_v7_0_gui.xml', @xlipmagiccallback_pass_evaluate_params, @xlipmagicaction)  CloseFcn=xlDestroyGui(gcbh);  MoveFcn=xlBlockMoveCallback(gcbh);
      mask Help: eval('');xlDoc('-book','sysgen','-topic','Fast_Fourier_Transform_7_0');
      mask StyleString: popup(8|16|32|64|128|256|512|1024|2048|4096|8192|16384|32768|65536),popup(automatically_select|pipelined_streaming_io|radix_4_burst_io|radix_2_burst_io|radix_2_lite_burst_io),edit,edit,checkbox,popup(8|9|10|11|12|13|14|15|16|17|18|19|20|21|22|23|24|25|26|27|28|29|30|31|32|33|34),popup(unscaled|scaled|block_floating_point),popup(truncation|convergent_rounding),popup(bit_reversed_order|natural_order),checkbox,checkbox,checkbox,checkbox,popup(no_offset|three_cycle_offset),popup(block_ram|distributed_ram),popup(block_ram|distributed_ram),popup(0|1|2|3|4|5|6|7|8|9|10|11),popup(block_ram|distributed_ram),checkbox,popup(use_luts|use_mults_resources|use_mults_performance),popup(use_luts|use_xtremedsp_slices),checkbox,edit,edit,edit,edit,edit,edit,edit,edit,edit,edit,edit,edit,edit,edit,edit,edit,edit,edit,edit,edit
      mask Display:
      | fprintf('','COMMENT: begin icon graphics');
      | patch([0 95 95 0 0 ],[0 0 142 142 0 ],[0.77 0.82 0.91 ]);
      | plot([0 95 95 0 0 ],[0 0 142 142 0 ]);
      | patch([18.075 36.86 49.86 62.86 75.86 49.86 31.075 18.075 ],[85.43 85.43 98.43 85.43 98.43 98.43 98.43 85.43 ],[1 1 1 ]);
      | patch([31.075 49.86 36.86 18.075 31.075 ],[72.43 72.43 85.43 85.43 72.43 ],[0.931 0.946 0.973 ]);
      | patch([18.075 36.86 49.86 31.075 18.075 ],[59.43 59.43 72.43 72.43 59.43 ],[1 1 1 ]);
      | patch([31.075 75.86 62.86 49.86 36.86 18.075 31.075 ],[46.43 46.43 59.43 46.43 59.43 59.43 46.43 ],[0.931 0.946 0.973 ]);
      | fprintf('','COMMENT: end icon graphics');
      | fprintf('','COMMENT: begin icon text');
      | color('black');port_label('input',1,'xn_re');
      | color('black');port_label('input',2,'xn_im');
      | color('black');port_label('input',3,'start');
      | color('black');port_label('input',4,'fwd_inv');
      | color('black');port_label('input',5,'fwd_inv_we');
      | color('black');port_label('input',6,'scale_sch');
      | color('black');port_label('input',7,'scale_sch_we');
      | color('black');port_label('output',1,'xk_re');
      | color('black');port_label('output',2,'xk_im');
      | color('black');port_label('output',3,'xn_index');
      | color('black');port_label('output',4,'xk_index');
      | color('black');port_label('output',5,'rfd');
      | color('black');port_label('output',6,'busy');
      | color('black');port_label('output',7,'dv');
      | color('black');port_label('output',8,'edone');
      | color('black');port_label('output',9,'done');
      | fprintf('','COMMENT: end icon text');
  "Fast Fourier Transform 7.1 " : S-Function  LoadFcn=xlBlockLoadCallback(gcbh);  FunctionName=sysgen  Parameters=ptable_  EnableBusSupport=off  mask(Xilinx Fast Fourier Transform 7.1 Block){transform_length=1024, implementation_options=pipelined_streaming_io, target_clock_frequency=250, target_data_throughput=50, run_time_configurable_transform_length=off, phase_factor_width=16, scaling_options=scaled, rounding_modes=truncation, output_ordering=bit_reversed_order, cyclic_prefix_insertion=off, ce=off, sclr=off, ovflo=off, input_data_offset=no_offset, memory_options_data=block_ram, memory_options_phase_factors=block_ram, number_of_stages_using_block_ram_for_data_and_phase_factors=1, memory_options_reorder=block_ram, memory_options_hybrid=off, complex_mult_type=use_mults_resources, butterfly_type=use_luts, xl_use_area=off, xl_area=[0,0,0,0,0,0,0], channels=1, input_ordering=natural_order, input_width=16, simulation_type=external_xfix, simulation_model=fftv71_CModel:fftv71_cmodel, ip_name=Fast Fourier Transform, ip_version=7.1, dsptool_ready=true, wrapper_available=true, port_translation_map={ 'ce' => 'en', 'sclr' => 'rst' }, ipcore_fpga_part=xlipgetpartsetting(gcb, {'virtex4', 'xc4vsx35', '-10', 'ff668'}), has_advanced_control=0, sggui_pos=-1,-1,-1,-1, block_type=xfft_v7_1, block_version=, sg_icon_stat=95,142,7,9,white,blue,0,c08fcb17,right,,[ ],[ ], sg_mask_display=|, sg_list_contents=, sg_blockgui_xml=}
      mask sg_mask_display=|
      | fprintf('','COMMENT: begin icon graphics');
      | patch([0 95 95 0 0 ],[0 0 142 142 0 ],[0.77 0.82 0.91 ]);
      | plot([0 95 95 0 0 ],[0 0 142 142 0 ]);
      | patch([18.075 36.86 49.86 62.86 75.86 49.86 31.075 18.075 ],[85.43 85.43 98.43 85.43 98.43 98.43 98.43 85.43 ],[1 1 1 ]);
      | patch([31.075 49.86 36.86 18.075 31.075 ],[72.43 72.43 85.43 85.43 72.43 ],[0.931 0.946 0.973 ]);
      | patch([18.075 36.86 49.86 31.075 18.075 ],[59.43 59.43 72.43 72.43 59.43 ],[1 1 1 ]);
      | patch([31.075 75.86 62.86 49.86 36.86 18.075 31.075 ],[46.43 46.43 59.43 46.43 59.43 59.43 46.43 ],[0.931 0.946 0.973 ]);
      | fprintf('','COMMENT: end icon graphics');
      | fprintf('','COMMENT: begin icon text');
      | color('black');port_label('input',1,'xn_re');
      | color('black');port_label('input',2,'xn_im');
      | color('black');port_label('input',3,'start');
      | color('black');port_label('input',4,'fwd_inv');
      | color('black');port_label('input',5,'fwd_inv_we');
      | color('black');port_label('input',6,'scale_sch');
      | color('black');port_label('input',7,'scale_sch_we');
      | color('black');port_label('output',1,'xk_re');
      | color('black');port_label('output',2,'xk_im');
      | color('black');port_label('output',3,'xn_index');
      | color('black');port_label('output',4,'xk_index');
      | color('black');port_label('output',5,'rfd');
      | color('black');port_label('output',6,'busy');
      | color('black');port_label('output',7,'dv');
      | color('black');port_label('output',8,'edone');
      | color('black');port_label('output',9,'done');
      | fprintf('','COMMENT: end icon text');
      mask prompts: transform_length ""; implementation_options ""; target_clock_frequency "Target clock frequency(MHz)"; target_data_throughput "Target data throughput(MSPS)"; run_time_configurable_transform_length "Run Time Configurable Transform Length"; phase_factor_width "Phase Factor Width"; scaling_options ""; rounding_modes ""; output_ordering ""; cyclic_prefix_insertion "Cyclic Prefix Insertion"; ce "en"; sclr "rst"; input_data_offset ""; memory_options_data ""; memory_options_phase_factors ""; number_of_stages_using_block_ram_for_data_and_phase_factors ""; memory_options_reorder ""; memory_options_hybrid "Optimize Block RAM count using hybrid memories"; complex_mult_type ""; butterfly_type ""; xl_use_area "Define FPGA area for resource estimation"; xl_area "FPGA area [slices, FFs, BRAMs, LUTs, IOBs, emb. mults, TBUFs]"; channels ""; input_ordering ""; input_width ""; simulation_type ""; simulation_model ""; ip_name ""; ip_version ""; dsptool_ready ""; wrapper_available ""; port_translation_map ""; ipcore_fpga_part ""; has_advanced_control ""; sggui_pos ""; block_type ""; block_version ""; sg_icon_stat ""; sg_mask_display ""; sg_list_contents ""; sg_blockgui_xml ""
      mask help: Xilinx Fast Fourier Transform 7.1
      mask init:
      | try
      |   tmp_gcb = gcb;
      |   tmp_gcbh = gcbh;
      |   if (strcmp('SysGenIndex',get_param(bdroot(tmp_gcbh),'tag')) && ~isempty(regexp(bdroot(tmp_gcb), '^xbs', 'once')))
      |     return;
      |   end;
      |   xlMungeMaskParams;
      |   block_config = 'sysgen:coregenimport_config';
      | 
      |   block_type='xfft_v7_1';
      | 
      |   serialized_declarations = '{''butterfly_type''=>''String'',''ce''=>''Bool'',''channels''=>''String'',''complex_mult_type''=>''String'',''cyclic_prefix_insertion''=>''Bool'',''dsptool_ready''=>''Bool'',''implementation_options''=>''String'',''input_data_offset''=>''String'',''input_ordering''=>''String'',''input_width''=>''String'',''ip_name''=>''String'',''ip_version''=>''String'',''ipcore_fpga_part''=>''StringVector'',''memory_options_data''=>''String'',''memory_options_hybrid''=>''Bool'',''memory_options_phase_factors''=>''String'',''memory_options_reorder''=>''String'',''number_of_stages_using_block_ram_for_data_and_phase_factors''=>''String'',''output_ordering''=>''String'',''ovflo''=>''Bool'',''phase_factor_width''=>''String'',''port_translation_map''=>''String'',''rounding_modes''=>''String'',''run_time_configurable_transform_length''=>''Bool'',''scaling_options''=>''String'',''sclr''=>''Bool'',''simulation_model''=>''String'',''simulation_type''=>''String'',''target_clock_frequency''=>''Int'',''target_data_throughput''=>''Int'',''transform_length''=>''String'',''wrapper_available''=>''Bool'',''xl_use_area''=>''Bool'',''block_type''=>''String''}';
      |   ptable_ = xlblockprep(get_param(tmp_gcb, 'MaskWSVariables'));
      |   try
      |     xlBlockMoveCallback(tmp_gcbh);
      |   catch 
      |      clear global xl_updateicon_recursion_guard;
      |   end;
      | catch
      |   global dbgsysgen;
      |   if(~isempty(dbgsysgen) && dbgsysgen)
      |     e = regexprep(lasterr, '\n', '\nError: ');
      |     disp(['Error: While running MaskInit code on block ' tmp_gcb ': ' e]);
      |     error(e);
      |   end
      | end
      settings: CopyFcn=xlBlockMoveCallback(gcbh);  DeleteFcn=xlDestroyGui(gcbh);  ModelCloseFcn=xlDestroyGui(gcbh);  PreSaveFcn=xlBlockPreSaveCallback(gcbh);  PostSaveFcn=xlBlockPostSaveCallback(gcbh);  DestroyFcn=xlDestroyGui(gcbh);  OpenFcn=xlOpenGui(gcbh, 'fft_v7_1_gui.xml', @xlipmagiccallback_pass_evaluate_params, @xlipmagicaction)  CloseFcn=xlDestroyGui(gcbh);  MoveFcn=xlBlockMoveCallback(gcbh);
      mask Help: eval('');xlDoc('-book','sysgen','-topic','Fast_Fourier_Transform_7_1');
      mask StyleString: popup(8|16|32|64|128|256|512|1024|2048|4096|8192|16384|32768|65536),popup(automatically_select|pipelined_streaming_io|radix_4_burst_io|radix_2_burst_io|radix_2_lite_burst_io),edit,edit,checkbox,popup(8|9|10|11|12|13|14|15|16|17|18|19|20|21|22|23|24|25|26|27|28|29|30|31|32|33|34),popup(unscaled|scaled|block_floating_point),popup(truncation|convergent_rounding),popup(bit_reversed_order|natural_order),checkbox,checkbox,checkbox,checkbox,popup(no_offset|three_cycle_offset),popup(block_ram|distributed_ram),popup(block_ram|distributed_ram),popup(0|1|2|3|4|5|6|7|8|9|10|11),popup(block_ram|distributed_ram),checkbox,popup(use_luts|use_mults_resources|use_mults_performance),popup(use_luts|use_xtremedsp_slices),checkbox,edit,edit,edit,edit,edit,edit,edit,edit,edit,edit,edit,edit,edit,edit,edit,edit,edit,edit,edit,edit
      mask Display:
      | fprintf('','COMMENT: begin icon graphics');
      | patch([0 95 95 0 0 ],[0 0 142 142 0 ],[0.77 0.82 0.91 ]);
      | plot([0 95 95 0 0 ],[0 0 142 142 0 ]);
      | patch([18.075 36.86 49.86 62.86 75.86 49.86 31.075 18.075 ],[85.43 85.43 98.43 85.43 98.43 98.43 98.43 85.43 ],[1 1 1 ]);
      | patch([31.075 49.86 36.86 18.075 31.075 ],[72.43 72.43 85.43 85.43 72.43 ],[0.931 0.946 0.973 ]);
      | patch([18.075 36.86 49.86 31.075 18.075 ],[59.43 59.43 72.43 72.43 59.43 ],[1 1 1 ]);
      | patch([31.075 75.86 62.86 49.86 36.86 18.075 31.075 ],[46.43 46.43 59.43 46.43 59.43 59.43 46.43 ],[0.931 0.946 0.973 ]);
      | fprintf('','COMMENT: end icon graphics');
      | fprintf('','COMMENT: begin icon text');
      | color('black');port_label('input',1,'xn_re');
      | color('black');port_label('input',2,'xn_im');
      | color('black');port_label('input',3,'start');
      | color('black');port_label('input',4,'fwd_inv');
      | color('black');port_label('input',5,'fwd_inv_we');
      | color('black');port_label('input',6,'scale_sch');
      | color('black');port_label('input',7,'scale_sch_we');
      | color('black');port_label('output',1,'xk_re');
      | color('black');port_label('output',2,'xk_im');
      | color('black');port_label('output',3,'xn_index');
      | color('black');port_label('output',4,'xk_index');
      | color('black');port_label('output',5,'rfd');
      | color('black');port_label('output',6,'busy');
      | color('black');port_label('output',7,'dv');
      | color('black');port_label('output',8,'edone');
      | color('black');port_label('output',9,'done');
      | fprintf('','COMMENT: end icon text');
  "Fast Fourier Transform 8.0 " : S-Function  LoadFcn=xlBlockLoadCallback(gcbh);  FunctionName=sysgen  Parameters=ptable_  EnableBusSupport=off  mask(Xilinx Fast Fourier Transform 8.0  Block){transform_length=1024, target_clock_frequency=250, target_data_throughput=50, implementation_options=pipelined_streaming_io, run_time_configurable_transform_length_sgadvanced=, run_time_configurable_transform_length=off, phase_factor_width=16, scaling_options_sgadvanced=, scaling_options=scaled, rounding_modes_sgadvanced=, rounding_modes=truncation, aclken_sgadvanced=, aclken=off, aresetn_sgadvanced=, aresetn=off, cyclic_prefix_insertion_sgadvanced=, cyclic_prefix_insertion=off, output_ordering_sgadvanced=, output_ordering=bit_reversed_order, throttle_scheme_sgadvanced=, throttle_scheme=nonrealtime, xk_index_sgadvanced=, xk_index=off, ovflo_sgadvanced=, ovflo=off, trim_axipin_name=on, memory_options_data_sgadvanced=, memory_options_data=block_ram, memory_options_phase_factors_sgadvanced=, memory_options_phase_factors=block_ram, number_of_stages_using_block_ram_for_data_and_phase_factors=1, memory_options_reorder_sgadvanced=, memory_options_reorder=block_ram, memory_options_hybrid_sgadvanced=, memory_options_hybrid=off, complex_mult_type_sgadvanced=, complex_mult_type=use_mults_resources, butterfly_type_sgadvanced=, butterfly_type=use_luts, xl_use_area=off, xl_area=[0,0,0,0,0,0,0], channels=1, input_ordering=natural_order, input_width=16, simulation_model=fftv8_CModel:fftv8_cmodel, ip_name=Fast Fourier Transform, ip_version=8.0, dsptool_ready=true, ipcore_usecache=true, ipcore_useipmodelcache=true, wrapper_available=true, port_translation_map={ 'aclken' => 'en', 'aresetn' => 'rst'}, has_advanced_control=0, sggui_pos=-1,-1,-1,-1, block_type=xfft_v8_0, block_version=, sg_icon_stat=225,250,8,12,white,blue,0,007d4553,right,,[2 2 2 3 3 3 3 4 ],[2 3 4 4 4 4 1 1 1 1 1 1 ], sg_mask_display=|, sg_list_contents=, sg_blockgui_xml=}
      mask sg_mask_display=|
      | fprintf('','COMMENT: begin icon graphics');
      | patch([0 0 4 4 ],[241 159 159 241 ],[6.025000e-001 6.400000e-001 7.075000e-001 ]);
      | patch([0 0 4 4 ],[151 39 39 151 ],[4.350000e-001 4.600000e-001 5.050000e-001 ]);
      | patch([0 0 4 4 ],[31 9 9 31 ],[2.675000e-001 2.800000e-001 3.025000e-001 ]);
      | patch([221 221 225 225 ],[242 228 228 242 ],[6.025000e-001 6.400000e-001 7.075000e-001 ]);
      | patch([221 221 225 225 ],[222 208 208 222 ],[4.350000e-001 4.600000e-001 5.050000e-001 ]);
      | patch([221 221 225 225 ],[202 128 128 202 ],[2.675000e-001 2.800000e-001 3.025000e-001 ]);
      | patch([221 221 225 225 ],[122 8 8 122 ],[7.700000e-001 8.200000e-001 9.100000e-001 ]);
      | patch([4 220 220 4 4 ],[0 0 250 250 0 ],[7.700000e-001 8.200000e-001 9.100000e-001 ]);
      | plot([4 220 220 4 4 ],[0 0 250 250 0 ]);
      |
      |
      | patch([40.8 87.04 119.04 151.04 183.04 119.04 72.8 40.8 ],[160.52 160.52 192.52 160.52 192.52 192.52 192.52 160.52 ],[1 1 1 ]);
      | patch([72.8 119.04 87.04 40.8 72.8 ],[128.52 128.52 160.52 160.52 128.52 ],[0.931 0.946 0.973 ]);
      | patch([40.8 87.04 119.04 72.8 40.8 ],[96.52 96.52 128.52 128.52 96.52 ],[1 1 1 ]);
      | patch([72.8 183.04 151.04 119.04 87.04 40.8 72.8 ],[64.52 64.52 96.52 64.52 96.52 96.52 64.52 ],[0.931 0.946 0.973 ]);
      | fprintf('','COMMENT: end icon graphics');
      | fprintf('','COMMENT: begin icon text');
      | color('black');port_label('input',1,'  config_tdata_scale_sch  ');
      | color('black');port_label('input',2,'  config_tdata_fwd_inv  ');
      | color('black');port_label('input',3,'  config_tvalid  ');
      | color('black');port_label('input',4,'  data_tdata_xn_im  ');
      | color('black');port_label('input',5,'  data_tdata_xn_re  ');
      | color('black');port_label('input',6,'  data_tvalid  ');
      | color('black');port_label('input',7,'  data_tlast  ');
      | color('black');port_label('input',8,'  data_tready  ');
      | color('black');port_label('output',1,'  config_tready  ');
      | color('black');port_label('output',2,'  data_tready  ');
      | color('black');port_label('output',3,'  data_tdata_xk_im  ');
      | color('black');port_label('output',4,'  data_tdata_xk_re  ');
      | color('black');port_label('output',5,'  data_tvalid  ');
      | color('black');port_label('output',6,'  data_tlast  ');
      | color('black');port_label('output',7,'  event_frame_started  ');
      | color('black');port_label('output',8,'  event_tlast_unexpected  ');
      | color('black');port_label('output',9,'  event_tlast_missing  ');
      | color('black');port_label('output',10,'  event_data_in_channel_halt  ');
      | color('black');port_label('output',11,'  event_status_channel_halt  ');
      | color('black');port_label('output',12,'  event_data_out_channel_halt  ');
      | fprintf('','COMMENT: end icon text');
      mask prompts: target_clock_frequency "Target Clock Frequency(MHz)"; target_data_throughput "Target Data Throughput(MSPS)"; implementation_options ""; run_time_configurable_transform_length_sgadvanced ""; run_time_configurable_transform_length "Run Time Configurable Transform Length"; phase_factor_width "Phase Factor Width"; scaling_options_sgadvanced ""; scaling_options ""; rounding_modes_sgadvanced ""; rounding_modes ""; aclken_sgadvanced ""; aresetn_sgadvanced ""; cyclic_prefix_insertion_sgadvanced ""; cyclic_prefix_insertion "Cyclic Prefix Insertion"; output_ordering_sgadvanced ""; output_ordering ""; throttle_scheme_sgadvanced ""; throttle_scheme ""; xk_index_sgadvanced ""; ovflo_sgadvanced ""; trim_axipin_name "Display shortened port names"; memory_options_data_sgadvanced ""; memory_options_data ""; memory_options_phase_factors_sgadvanced ""; memory_options_phase_factors ""; number_of_stages_using_block_ram_for_data_and_phase_factors ""; memory_options_reorder_sgadvanced ""; memory_options_reorder ""; memory_options_hybrid_sgadvanced ""; memory_options_hybrid "Optimize Block RAM Count Using Hybrid Memories"; complex_mult_type_sgadvanced ""; complex_mult_type ""; butterfly_type_sgadvanced ""; butterfly_type ""; xl_use_area "Define FPGA area for resource estimation"; xl_area "FPGA area [slices, FFs, BRAMs, LUTs, IOBs, emb. mults, TBUFs]"; channels ""; input_ordering ""; input_width ""; simulation_model ""; ip_name ""; ip_version ""; dsptool_ready ""; ipcore_usecache ""; ipcore_useipmodelcache ""; wrapper_available ""; port_translation_map ""; has_advanced_control ""; sggui_pos ""; block_type ""; block_version ""; sg_icon_stat ""; sg_mask_display ""; sg_list_contents ""; sg_blockgui_xml ""
      mask help: Xilinx Fast Fourier Transform 8.0
      mask init:
      | try
      |   tmp_gcb = gcb;
      |   tmp_gcbh = gcbh;
      |   if (strcmp('SysGenIndex',get_param(bdroot(tmp_gcbh),'tag')) && ~isempty(regexp(bdroot(tmp_gcb), '^xbs', 'once')))
      |     return;
      |   end;
      |   xlMungeMaskParams;
      |   block_config = 'sysgen:coregenimport_config';
      | 
      |   block_type='xfft_v8_0';
      | 
      |   serialized_declarations = '{''aclken''=>''Bool'',''aresetn''=>''Bool'',''butterfly_type''=>''String'',''channels''=>''String'',''complex_mult_type''=>''String'',''cyclic_prefix_insertion''=>''Bool'',''dsptool_ready''=>''Bool'',''implementation_options''=>''String'',''input_ordering''=>''String'',''input_width''=>''String'',''ip_name''=>''String'',''ip_version''=>''String'',''ipcore_usecache''=>''Bool'',''ipcore_useipmodelcache''=>''Bool'',''memory_options_data''=>''String'',''memory_options_hybrid''=>''Bool'',''memory_options_phase_factors''=>''String'',''memory_options_reorder''=>''String'',''number_of_stages_using_block_ram_for_data_and_phase_factors''=>''String'',''output_ordering''=>''String'',''ovflo''=>''Bool'',''phase_factor_width''=>''String'',''port_translation_map''=>''String'',''rounding_modes''=>''String'',''run_time_configurable_transform_length''=>''Bool'',''scaling_options''=>''String'',''simulation_model''=>''String'',''simulation_type''=>''String'',''target_clock_frequency''=>''Int'',''target_data_throughput''=>''Int'',''throttle_scheme''=>''String'',''transform_length''=>''String'',''trim_axipin_name''=>''Int'',''wrapper_available''=>''Bool'',''xk_index''=>''Bool'',''xl_use_area''=>''Bool'',''block_type''=>''String''}';
      |   xlfftv8_init();
      |   ptable_ = xlblockprep(get_param(tmp_gcb, 'MaskWSVariables'));
      |   try
      |     xlBlockMoveCallback(tmp_gcbh);
      |   catch 
      |      clear global xl_updateicon_recursion_guard;
      |   end;
      | catch
      |   global dbgsysgen;
      |   if(~isempty(dbgsysgen) && dbgsysgen)
      |     e = regexprep(lasterr, '\n', '\nError: ');
      |     disp(['Error: While running MaskInit code on block ' tmp_gcb ': ' e]);
      |     error(e);
      |   end
      | end
      settings: CopyFcn=xlBlockMoveCallback(gcbh);  DeleteFcn=xlDestroyGui(gcbh);  ModelCloseFcn=xlDestroyGui(gcbh);  PreSaveFcn=xlBlockPreSaveCallback(gcbh);  PostSaveFcn=xlBlockPostSaveCallback(gcbh);  DestroyFcn=xlDestroyGui(gcbh);  OpenFcn=xlOpenGui(gcbh, 'fft_v8_0_gui.xml', @xlipmagiccallback_pass_evaluate_params, @xlipmagicaction)  CloseFcn=xlDestroyGui(gcbh);  MoveFcn=xlBlockMoveCallback(gcbh);
      mask Help: eval('');xlDoc('-book','sysgen','-topic','Fast_Fourier_Transform_8_0');
      mask StyleString: popup(8|16|32|64|128|256|512|1024|2048|4096|8192|16384|32768|65536),edit,edit,popup(automatically_select|pipelined_streaming_io|radix_4_burst_io|radix_2_burst_io|radix_2_lite_burst_io),edit,checkbox,popup(8|9|10|11|12|13|14|15|16|17|18|19|20|21|22|23|24|25|26|27|28|29|30|31|32|33|34),edit,popup(unscaled|scaled|block_floating_point),edit,popup(truncation|convergent_rounding),edit,checkbox,edit,checkbox,edit,checkbox,edit,popup(bit_reversed_order|natural_order),edit,popup(realtime|nonrealtime),edit,checkbox,edit,checkbox,checkbox,edit,popup(block_ram|distributed_ram),edit,popup(block_ram|distributed_ram),popup(0|1|2|3|4|5|6|7|8|9|10|11),edit,popup(block_ram|distributed_ram),edit,checkbox,edit,popup(use_luts|use_mults_resources|use_mults_performance),edit,popup(use_luts|use_xtremedsp_slices),checkbox,edit,edit,edit,edit,edit,edit,edit,edit,edit,edit,edit,edit,edit,edit,edit,edit,edit,edit,edit,edit
      mask Display:
      | fprintf('','COMMENT: begin icon graphics');
      | patch([0 0 4 4 ],[241 159 159 241 ],[6.025000e-001 6.400000e-001 7.075000e-001 ]);
      | patch([0 0 4 4 ],[151 39 39 151 ],[4.350000e-001 4.600000e-001 5.050000e-001 ]);
      | patch([0 0 4 4 ],[31 9 9 31 ],[2.675000e-001 2.800000e-001 3.025000e-001 ]);
      | patch([221 221 225 225 ],[242 228 228 242 ],[6.025000e-001 6.400000e-001 7.075000e-001 ]);
      | patch([221 221 225 225 ],[222 208 208 222 ],[4.350000e-001 4.600000e-001 5.050000e-001 ]);
      | patch([221 221 225 225 ],[202 128 128 202 ],[2.675000e-001 2.800000e-001 3.025000e-001 ]);
      | patch([221 221 225 225 ],[122 8 8 122 ],[7.700000e-001 8.200000e-001 9.100000e-001 ]);
      | patch([4 220 220 4 4 ],[0 0 250 250 0 ],[7.700000e-001 8.200000e-001 9.100000e-001 ]);
      | plot([4 220 220 4 4 ],[0 0 250 250 0 ]);
      | 
      | 
      | patch([40.8 87.04 119.04 151.04 183.04 119.04 72.8 40.8 ],[160.52 160.52 192.52 160.52 192.52 192.52 192.52 160.52 ],[1 1 1 ]);
      | patch([72.8 119.04 87.04 40.8 72.8 ],[128.52 128.52 160.52 160.52 128.52 ],[0.931 0.946 0.973 ]);
      | patch([40.8 87.04 119.04 72.8 40.8 ],[96.52 96.52 128.52 128.52 96.52 ],[1 1 1 ]);
      | patch([72.8 183.04 151.04 119.04 87.04 40.8 72.8 ],[64.52 64.52 96.52 64.52 96.52 96.52 64.52 ],[0.931 0.946 0.973 ]);
      | fprintf('','COMMENT: end icon graphics');
      | fprintf('','COMMENT: begin icon text');
      | color('black');port_label('input',1,'  config_tdata_scale_sch  ');
      | color('black');port_label('input',2,'  config_tdata_fwd_inv  ');
      | color('black');port_label('input',3,'  config_tvalid  ');
      | color('black');port_label('input',4,'  data_tdata_xn_im  ');
      | color('black');port_label('input',5,'  data_tdata_xn_re  ');
      | color('black');port_label('input',6,'  data_tvalid  ');
      | color('black');port_label('input',7,'  data_tlast  ');
      | color('black');port_label('input',8,'  data_tready  ');
      | color('black');port_label('output',1,'  config_tready  ');
      | color('black');port_label('output',2,'  data_tready  ');
      | color('black');port_label('output',3,'  data_tdata_xk_im  ');
      | color('black');port_label('output',4,'  data_tdata_xk_re  ');
      | color('black');port_label('output',5,'  data_tvalid  ');
      | color('black');port_label('output',6,'  data_tlast  ');
      | color('black');port_label('output',7,'  event_frame_started  ');
      | color('black');port_label('output',8,'  event_tlast_unexpected  ');
      | color('black');port_label('output',9,'  event_tlast_missing  ');
      | color('black');port_label('output',10,'  event_data_in_channel_halt  ');
      | color('black');port_label('output',11,'  event_status_channel_halt  ');
      | color('black');port_label('output',12,'  event_data_out_channel_halt  ');
      | fprintf('','COMMENT: end icon text');
  From FIFO : S-Function  LoadFcn=xlBlockLoadCallback(gcbh);  FunctionName=sysgen  Parameters=ptable_  EnableBusSupport=off  mask(Xilinx Shared Memory Based From FIFO Block){infoedit=First-in-first-out (FIFO) block that reads FIFO data from shared memory storage., shared_memory_name='Bar', ownership_sgadvanced=, ownership=Owned elsewhere, performance_options_sgadvanced=, performance_options=Standard_FIFO, depth_sgadvanced=, depth=16, percent_nbits_sgadvanced=, percent_nbits=1, has_arst_sgadvanced=, has_arst=off, use_percent_full_port_sgadvanced=, use_percent_full_port=on, gui_display_data_type=Fixed-point, arith_type_sgadvanced=, arith_type=Signed  (2's comp), n_bits=16, bin_pt=14, preci_type_sgadvanced=, preci_type=Single, dbl_ovrd_sgadvanced=, dbl_ovrd=off, mem_type_sgadvanced=, mem_type=Block RAM, xl_use_area_sgadvanced=, xl_use_area=off, xl_area=[0,0,0,0,0,0,0], has_advanced_control=0, sggui_pos=-1,-1,-1,-1, block_type=fromfifo, block_version=, sg_icon_stat=80,90,1,3,white,blue,0,ddb0a084,right,,[ ],[ ], sg_mask_display=|, sg_list_contents=, sg_blockgui_xml=}
      mask sg_mask_display=|
      | fprintf('','COMMENT: begin icon graphics');
      | patch([0 80 80 0 0 ],[0 0 90 90 0 ],[0.77 0.82 0.91 ]);
      | plot([0 80 80 0 0 ],[0 0 90 90 0 ]);
      | patch([15.525 31.42 42.42 53.42 64.42 42.42 26.525 15.525 ],[57.21 57.21 68.21 57.21 68.21 68.21 68.21 57.21 ],[1 1 1 ]);
      | patch([26.525 42.42 31.42 15.525 26.525 ],[46.21 46.21 57.21 57.21 46.21 ],[0.931 0.946 0.973 ]);
      | patch([15.525 31.42 42.42 26.525 15.525 ],[35.21 35.21 46.21 46.21 35.21 ],[1 1 1 ]);
      | patch([26.525 64.42 53.42 42.42 31.42 15.525 26.525 ],[24.21 24.21 35.21 24.21 35.21 35.21 24.21 ],[0.931 0.946 0.973 ]);
      | fprintf('','COMMENT: end icon graphics');
      | fprintf('','COMMENT: begin icon text');
      | color('black');port_label('input',1,'re');
      | color('black');port_label('output',1,'dout');
      | color('black');port_label('output',2,'%full');
      | color('black');port_label('output',3,'empty');
      | fprintf('','COMMENT: end icon text');
      mask prompts: infoedit ""; shared_memory_name "Shared memory name"; ownership_sgadvanced ""; performance_options_sgadvanced ""; performance_options "Performance Options"; depth_sgadvanced ""; percent_nbits_sgadvanced ""; percent_nbits "Bits of precision to use for <tt>%full</tt> port"; has_arst_sgadvanced ""; has_arst "Provide asynchronous reset port"; use_percent_full_port_sgadvanced ""; use_percent_full_port "Provide percent full port"; gui_display_data_type ""; arith_type_sgadvanced ""; arith_type "Arithmetic type"; n_bits "Number of bits"; bin_pt "Binary point"; preci_type_sgadvanced ""; preci_type ""; dbl_ovrd_sgadvanced ""; dbl_ovrd "Override with doubles"; mem_type_sgadvanced ""; mem_type "Memory Type"; xl_use_area_sgadvanced ""; xl_use_area "Define FPGA area for resource estimation"; xl_area "FPGA area [slices, FFs, BRAMs, LUTs, IOBs, emb. mults, TBUFs]"; has_advanced_control ""; sggui_pos ""; block_type ""; block_version ""; sg_icon_stat ""; sg_mask_display ""; sg_list_contents ""; sg_blockgui_xml ""
      mask help: First-in-first-out (FIFO) block that reads FIFO data from shared memory storage.
      mask init:
      | try
      |   tmp_gcb = gcb;
      |   tmp_gcbh = gcbh;
      |   if (strcmp('SysGenIndex',get_param(bdroot(tmp_gcbh),'tag')) && ~isempty(regexp(bdroot(tmp_gcb), '^xbs', 'once')))
      |     return;
      |   end;
      |   xlMungeMaskParams;
      |   block_config = 'sysgen_blockset:fromfifo_config';
      | 
      |   block_type='fromfifo';
      | 
      |   serialized_declarations = '{''arith_type''=>''Int'',''bin_pt''=>''Int'',''dbl_ovrd''=>''Int'',''depth''=>''Int'',''gui_display_data_type''=>''Int'',''has_arst''=>''Int'',''mem_type''=>''Int'',''n_bits''=>''Int'',''ownership''=>''Int'',''percent_nbits''=>''Int'',''performance_options''=>''Int'',''preci_type''=>''Int'',''shared_memory_name''=>''String'',''use_percent_full_port''=>''Int'',''block_type''=>''String''}';
      |   ptable_ = xlblockprep(get_param(tmp_gcb, 'MaskWSVariables'));
      |   try
      |     xlBlockMoveCallback(tmp_gcbh);
      |   catch 
      |      clear global xl_updateicon_recursion_guard;
      |   end;
      | catch
      |   global dbgsysgen;
      |   if(~isempty(dbgsysgen) && dbgsysgen)
      |     e = regexprep(lasterr, '\n', '\nError: ');
      |     disp(['Error: While running MaskInit code on block ' tmp_gcb ': ' e]);
      |     error(e);
      |   end
      | end
      settings: AttributesFormatString=<< %<shared_memory_name> >>  CopyFcn=xlBlockMoveCallback(gcbh);  DeleteFcn=xlDestroyGui(gcbh);  ModelCloseFcn=xlDestroyGui(gcbh);  PreSaveFcn=xlBlockPreSaveCallback(gcbh);  PostSaveFcn=xlBlockPostSaveCallback(gcbh);  DestroyFcn=xlDestroyGui(gcbh);  OpenFcn=xlOpenGui(gcbh, 'fromfifo_gui.xml', @fromfifoenablement, @xlDatatypeAction)  CloseFcn=xlDestroyGui(gcbh);  MoveFcn=xlBlockMoveCallback(gcbh);
      mask Help: eval('');xlDoc('-book','sysgen','-topic','From_FIFO');
      mask StyleString: edit,edit,edit,popup(Locally owned|Owned elsewhere),edit,popup(Standard_FIFO|First_Word_Fall_Through),edit,popup(16|32|64|128|256|512|1K|2K|4K|8K|16K|32K|64K|128K|256K),edit,popup(1|2|3|4|5|6|7|8|9|10|11|12|13|14|15|16|17|18),edit,checkbox,edit,checkbox,popup(Fixed-point|Floating-point),edit,popup(Signed  (2's comp)|Unsigned|Floating-point),edit,edit,edit,popup(Single),edit,checkbox,edit,popup(Block RAM|Distributed RAM),edit,checkbox,edit,edit,edit,edit,edit,edit,edit,edit,edit
      mask Display:
      | fprintf('','COMMENT: begin icon graphics');
      | patch([0 80 80 0 0 ],[0 0 90 90 0 ],[0.77 0.82 0.91 ]);
      | plot([0 80 80 0 0 ],[0 0 90 90 0 ]);
      | patch([15.525 31.42 42.42 53.42 64.42 42.42 26.525 15.525 ],[57.21 57.21 68.21 57.21 68.21 68.21 68.21 57.21 ],[1 1 1 ]);
      | patch([26.525 42.42 31.42 15.525 26.525 ],[46.21 46.21 57.21 57.21 46.21 ],[0.931 0.946 0.973 ]);
      | patch([15.525 31.42 42.42 26.525 15.525 ],[35.21 35.21 46.21 46.21 35.21 ],[1 1 1 ]);
      | patch([26.525 64.42 53.42 42.42 31.42 15.525 26.525 ],[24.21 24.21 35.21 24.21 35.21 35.21 24.21 ],[0.931 0.946 0.973 ]);
      | fprintf('','COMMENT: end icon graphics');
      | fprintf('','COMMENT: begin icon text');
      | color('black');port_label('input',1,'re');
      | color('black');port_label('output',1,'dout');
      | color('black');port_label('output',2,'%full');
      | color('black');port_label('output',3,'empty');
      | fprintf('','COMMENT: end icon text');
  From Register : S-Function  LoadFcn=xlBlockLoadCallback(gcbh);  FunctionName=sysgen  Parameters=ptable_  EnableBusSupport=off  mask(Xilinx Shared Memory Based From Register Block){infoedit=Register block that reads data to a shared memory register.  Delay of one sample period., shared_memory_name='Bar', init=0, period=1, ownership_sgadvanced=, ownership=Owned and initialized elsewhere, gui_display_data_type=Fixed-point, arith_type_sgadvanced=, arith_type=Signed  (2's comp), n_bits=16, bin_pt=14, preci_type_sgadvanced=, preci_type=Single, dbl_ovrd_sgadvanced=, dbl_ovrd=off, xl_use_area_sgadvanced=, xl_use_area=off, xl_area=[0,0,0,0,0,0,0], has_advanced_control=0, sggui_pos=-1,-1,-1,-1, block_type=fromreg, block_version=, sg_icon_stat=60,56,0,1,white,blue,0,b27a07ff,right,,[ ],[ ], sg_mask_display=|, sg_list_contents=, sg_blockgui_xml=}
      mask sg_mask_display=|
      | fprintf('','COMMENT: begin icon graphics');
      | patch([0 60 60 0 0 ],[0 0 56 56 0 ],[0.77 0.82 0.91 ]);
      | plot([0 60 60 0 0 ],[0 0 56 56 0 ]);
      | patch([12.2 23.76 31.76 39.76 47.76 31.76 20.2 12.2 ],[36.88 36.88 44.88 36.88 44.88 44.88 44.88 36.88 ],[1 1 1 ]);
      | patch([20.2 31.76 23.76 12.2 20.2 ],[28.88 28.88 36.88 36.88 28.88 ],[0.931 0.946 0.973 ]);
      | patch([12.2 23.76 31.76 20.2 12.2 ],[20.88 20.88 28.88 28.88 20.88 ],[1 1 1 ]);
      | patch([20.2 47.76 39.76 31.76 23.76 12.2 20.2 ],[12.88 12.88 20.88 12.88 20.88 20.88 12.88 ],[0.931 0.946 0.973 ]);
      | fprintf('','COMMENT: end icon graphics');
      | fprintf('','COMMENT: begin icon text');
      | color('black');port_label('output',1,'dout');
      | fprintf('','COMMENT: end icon text');
      mask prompts: infoedit ""; shared_memory_name "Shared memory name"; init "Initial value"; period "Sample period"; ownership_sgadvanced ""; ownership "Ownership and initialization"; gui_display_data_type ""; arith_type_sgadvanced ""; arith_type "Arithmetic type"; n_bits "Number of bits"; bin_pt "Binary point"; preci_type_sgadvanced ""; preci_type ""; dbl_ovrd_sgadvanced ""; dbl_ovrd "Override with doubles"; xl_use_area_sgadvanced ""; xl_use_area "Define FPGA area for resource estimation"; xl_area "FPGA area [slices, FFs, BRAMs, LUTs, IOBs, emb. mults, TBUFs]"; has_advanced_control ""; sggui_pos ""; block_type ""; block_version ""; sg_icon_stat ""; sg_mask_display ""; sg_list_contents ""; sg_blockgui_xml ""
      mask help: Register block that reads data to a shared memory register. Delay of one sample period.
      mask init:
      | try
      |   tmp_gcb = gcb;
      |   tmp_gcbh = gcbh;
      |   if (strcmp('SysGenIndex',get_param(bdroot(tmp_gcbh),'tag')) && ~isempty(regexp(bdroot(tmp_gcb), '^xbs', 'once')))
      |     return;
      |   end;
      |   xlMungeMaskParams;
      |   block_config = 'sysgen_blockset:fromreg_config';
      | 
      |   block_type='fromreg';
      | 
      |   serialized_declarations = '{''arith_type''=>''Int'',''bin_pt''=>''Int'',''dbl_ovrd''=>''Int'',''gui_display_data_type''=>''Int'',''init''=>''Double'',''n_bits''=>''Int'',''ownership''=>''Int'',''period''=>''Double'',''preci_type''=>''Int'',''shared_memory_name''=>''String'',''block_type''=>''String''}';
      |   ptable_ = xlblockprep(get_param(tmp_gcb, 'MaskWSVariables'));
      |   try
      |     xlBlockMoveCallback(tmp_gcbh);
      |   catch 
      |      clear global xl_updateicon_recursion_guard;
      |   end;
      | catch
      |   global dbgsysgen;
      |   if(~isempty(dbgsysgen) && dbgsysgen)
      |     e = regexprep(lasterr, '\n', '\nError: ');
      |     disp(['Error: While running MaskInit code on block ' tmp_gcb ': ' e]);
      |     error(e);
      |   end
      | end
      settings: AttributesFormatString=<< %<shared_memory_name> >>  CopyFcn=xlBlockMoveCallback(gcbh);  DeleteFcn=xlDestroyGui(gcbh);  ModelCloseFcn=xlDestroyGui(gcbh);  PreSaveFcn=xlBlockPreSaveCallback(gcbh);  PostSaveFcn=xlBlockPostSaveCallback(gcbh);  DestroyFcn=xlDestroyGui(gcbh);  OpenFcn=xlOpenGui(gcbh, 'fromreg_gui.xml', @fromregenablement, @xlDatatypeAction)  CloseFcn=xlDestroyGui(gcbh);  MoveFcn=xlBlockMoveCallback(gcbh);
      mask Help: eval('');xlDoc('-book','sysgen','-topic','From_Register');
      mask StyleString: edit,edit,edit,edit,edit,popup(Locally owned and initialized|Owned and initialized elsewhere),popup(Fixed-point|Floating-point),edit,popup(Signed  (2's comp)|Unsigned|Floating-point),edit,edit,edit,popup(Single),edit,checkbox,edit,checkbox,edit,edit,edit,edit,edit,edit,edit,edit,edit
      mask Display:
      | fprintf('','COMMENT: begin icon graphics');
      | patch([0 60 60 0 0 ],[0 0 56 56 0 ],[0.77 0.82 0.91 ]);
      | plot([0 60 60 0 0 ],[0 0 56 56 0 ]);
      | patch([12.2 23.76 31.76 39.76 47.76 31.76 20.2 12.2 ],[36.88 36.88 44.88 36.88 44.88 44.88 44.88 36.88 ],[1 1 1 ]);
      | patch([20.2 31.76 23.76 12.2 20.2 ],[28.88 28.88 36.88 36.88 28.88 ],[0.931 0.946 0.973 ]);
      | patch([12.2 23.76 31.76 20.2 12.2 ],[20.88 20.88 28.88 28.88 20.88 ],[1 1 1 ]);
      | patch([20.2 47.76 39.76 31.76 23.76 12.2 20.2 ],[12.88 12.88 20.88 12.88 20.88 20.88 12.88 ],[0.931 0.946 0.973 ]);
      | fprintf('','COMMENT: end icon graphics');
      | fprintf('','COMMENT: begin icon text');
      | color('black');port_label('output',1,'dout');
      | fprintf('','COMMENT: end icon text');
  Gateway In : S-Function  LoadFcn=xlBlockLoadCallback(gcbh);  FunctionName=sysgen  Parameters=ptable_  EnableBusSupport=off  mask(Xilinx Gateway In Block){infoedit=Gateway in block.  Converts inputs of type Simulink integer, single, double and fixed point to  Xilinx fixed-point or floating-point data type.<br><br>Hardware notes:  In hardware these blocks become top level input ports., gui_display_data_type_sgadvanced=, gui_display_data_type=Fixed-point, arith_type_sgadvanced=, arith_type=Signed  (2's comp), n_bits=16, bin_pt=14, preci_type_sgadvanced=, preci_type=Single, exp_width=8, frac_width=24, quantization_sgadvanced=, quantization=Round  (unbiased: +/- Inf), overflow_sgadvanced=, overflow=Saturate, period=1, dbl_ovrd_sgadvanced=, dbl_ovrd=off, timing_constraint_sgadvanced=, timing_constraint=None, locs_specified_sgadvanced=, locs_specified=off, LOCs={}, xl_use_area_sgadvanced=, xl_use_area=off, xl_area=[0,0,0,0,0,0,0], inherit_from_input_sgadvanced=, inherit_from_input=off, UseAsADC_sgadvanced=, UseAsADC=off, ADCChannel='1', hdl_port=on, sginterface=, has_advanced_control=0, sggui_pos=-1,-1,-1,-1, block_type=gatewayin, block_version=, sg_icon_stat=65,20,1,1,white,yellow,1,00d3666e,right,,[ ],[ ], sg_mask_display=|, sg_list_contents=, sg_blockgui_xml=}
      mask sg_mask_display=|
      | fprintf('','COMMENT: begin icon graphics');
      | patch([0 65 65 0 0 ],[0 0 20 20 0 ],[0.95 0.93 0.65 ]);
      | plot([0 65 65 0 0 ],[0 0 20 20 0 ]);
      | patch([27.55 30.44 32.44 34.44 36.44 32.44 29.55 27.55 ],[12.22 12.22 14.22 12.22 14.22 14.22 14.22 12.22 ],[1 1 1 ]);
      | patch([29.55 32.44 30.44 27.55 29.55 ],[10.22 10.22 12.22 12.22 10.22 ],[0.985 0.979 0.895 ]);
      | patch([27.55 30.44 32.44 29.55 27.55 ],[8.22 8.22 10.22 10.22 8.22 ],[1 1 1 ]);
      | patch([29.55 36.44 34.44 32.44 30.44 27.55 29.55 ],[6.22 6.22 8.22 6.22 8.22 8.22 6.22 ],[0.985 0.979 0.895 ]);
      | fprintf('','COMMENT: end icon graphics');
      | fprintf('','COMMENT: begin icon text');
      | color('black');port_label('input',1,'\fontsize{11pt}\bf In ','texmode','on');
      | color('black');port_label('output',1,' ');
      | fprintf('','COMMENT: end icon text');
      mask prompts: infoedit ""; gui_display_data_type_sgadvanced ""; gui_display_data_type ""; arith_type_sgadvanced ""; arith_type "Arithmetic type"; n_bits "Number of bits"; bin_pt "Binary point"; preci_type_sgadvanced ""; preci_type ""; exp_width "Exponent width"; frac_width "Fraction width"; quantization_sgadvanced ""; overflow_sgadvanced ""; period "Sample period"; dbl_ovrd_sgadvanced ""; dbl_ovrd "Override with doubles"; timing_constraint_sgadvanced ""; timing_constraint "IOB timing constraint"; locs_specified_sgadvanced ""; locs_specified "Specify IOB location constraints"; LOCs "IOB pad locations (specify as cell array {'MSB', ..., 'LSB'})"; xl_use_area_sgadvanced ""; xl_use_area "Define FPGA area for resource estimation"; xl_area "FPGA area [slices, FFs, BRAMs, LUTs, IOBs, emb. mults, TBUFs]"; inherit_from_input_sgadvanced ""; inherit_from_input "Inherit from input"; UseAsADC_sgadvanced ""; UseAsADC "Use ADC Input"; ADCChannel "ADC Channel ID"; hdl_port ""; sginterface ""; has_advanced_control ""; sggui_pos ""; block_type ""; block_version ""; sg_icon_stat ""; sg_mask_display ""; sg_list_contents ""; sg_blockgui_xml ""
      mask help:
      | Gateway in block.  Converts inputs of type Simulink integer, single, double and fixed point to  Xilinx fixed-point or floating-point data type.
      |
      | Hardware notes:  In hardware these blocks become top level input ports.
      mask init:
      | try
      |   tmp_gcb = gcb;
      |   tmp_gcbh = gcbh;
      |   if (strcmp('SysGenIndex',get_param(bdroot(tmp_gcbh),'tag')) && ~isempty(regexp(bdroot(tmp_gcb), '^xbs', 'once')))
      |     return;
      |   end;
      |   xlMungeMaskParams;
      |   block_config = 'sysgen_blockset:gateway_in_config';
      | 
      |   block_type='gatewayin';
      | 
      |   serialized_declarations = '{''ADCChannel''=>''String'',''LOCs''=>''StringVector'',''UseAsADC''=>''Int'',''arith_type''=>''Int'',''bin_pt''=>''Int'',''exp_width''=>''Int'',''frac_width''=>''Int'',''gui_display_data_type''=>''Int'',''hdl_port''=>''String'',''inherit_from_input''=>''Int'',''locs_specified''=>''Int'',''n_bits''=>''Int'',''overflow''=>''Int'',''period''=>''Double'',''preci_type''=>''Int'',''quantization''=>''Int'',''sginterface''=>''String'',''timing_constraint''=>''Int'',''block_type''=>''String''}';
      |   ptable_ = xlblockprep(get_param(tmp_gcb, 'MaskWSVariables'));
      |   try
      |     xlBlockMoveCallback(tmp_gcbh);
      |   catch 
      |      clear global xl_updateicon_recursion_guard;
      |   end;
      | catch
      |   global dbgsysgen;
      |   if(~isempty(dbgsysgen) && dbgsysgen)
      |     e = regexprep(lasterr, '\n', '\nError: ');
      |     disp(['Error: While running MaskInit code on block ' tmp_gcb ': ' e]);
      |     error(e);
      |   end
      | end
      settings: CopyFcn=xlBlockMoveCallback(gcbh);  DeleteFcn=xlDestroyGui(gcbh);  ModelCloseFcn=xlDestroyGui(gcbh);  PreSaveFcn=xlBlockPreSaveCallback(gcbh);  PostSaveFcn=xlBlockPostSaveCallback(gcbh);  DestroyFcn=xlDestroyGui(gcbh);  OpenFcn=xlOpenGui(gcbh, 'gatewayin_gui.xml', @gatewayinenablement, @gatewayinaction)  CloseFcn=xlDestroyGui(gcbh);  MoveFcn=xlBlockMoveCallback(gcbh);
      mask Help: eval('');xlDoc('-book','sysgen','-topic','Gateway_In');
      mask StyleString: edit,edit,popup(Boolean|Fixed-point|Floating-point),edit,popup(Boolean|Signed  (2's comp)|Unsigned|Floating-point),edit,edit,edit,popup(Single|Double|Custom),edit,edit,edit,popup(Truncate|Round  (unbiased: +/- Inf)),edit,popup(Wrap|Saturate|Flag as error),edit,edit,checkbox,edit,popup(None|Data Rate),edit,checkbox,edit,edit,checkbox,edit,edit,checkbox,edit,checkbox,edit,edit,edit,edit,edit,edit,edit,edit,edit,edit,edit
      mask Display:
      | fprintf('','COMMENT: begin icon graphics');
      | patch([0 65 65 0 0 ],[0 0 20 20 0 ],[0.95 0.93 0.65 ]);
      | plot([0 65 65 0 0 ],[0 0 20 20 0 ]);
      | patch([27.55 30.44 32.44 34.44 36.44 32.44 29.55 27.55 ],[12.22 12.22 14.22 12.22 14.22 14.22 14.22 12.22 ],[1 1 1 ]);
      | patch([29.55 32.44 30.44 27.55 29.55 ],[10.22 10.22 12.22 12.22 10.22 ],[0.985 0.979 0.895 ]);
      | patch([27.55 30.44 32.44 29.55 27.55 ],[8.22 8.22 10.22 10.22 8.22 ],[1 1 1 ]);
      | patch([29.55 36.44 34.44 32.44 30.44 27.55 29.55 ],[6.22 6.22 8.22 6.22 8.22 8.22 6.22 ],[0.985 0.979 0.895 ]);
      | fprintf('','COMMENT: end icon graphics');
      | fprintf('','COMMENT: begin icon text');
      | color('black');port_label('input',1,'\fontsize{11pt}\bf In ','texmode','on');
      | color('black');port_label('output',1,' ');
      | fprintf('','COMMENT: end icon text');
  Gateway Out : S-Function  LoadFcn=xlBlockLoadCallback(gcbh);  FunctionName=sysgen  Parameters=ptable_  EnableBusSupport=off  mask(Xilinx Gateway Out Block){infoedit=Gateway out block.  Converts Xilinx fixed-point or floating-point type inputs into ouputs of type Simulink integer, single, double, or fixed point.<br><br>Hardware notes:  In hardware these blocks become top level output ports or are discarded, depending on how they are configured., inherit_from_input_sgadvanced=, inherit_from_input=off, hdl_port_sgadvanced=, hdl_port=on, timing_constraint_sgadvanced=, timing_constraint=None, locs_specified_sgadvanced=, locs_specified=off, LOCs={}, xl_use_area_sgadvanced=, xl_use_area=off, xl_area=[0,0,0,0,0,0,0], UseAsDAC_sgadvanced=, UseAsDAC=off, DACChannel='1', sginterface=, has_advanced_control=0, sggui_pos=-1,-1,-1,-1, block_type=gatewayout, block_version=, sg_icon_stat=60,20,1,1,white,yellow,1,cc31b7ac,right,,[ ],[ ], sg_mask_display=|, sg_list_contents=, sg_blockgui_xml=}
      mask sg_mask_display=|
      | fprintf('','COMMENT: begin icon graphics');
      | patch([0 60 60 0 0 ],[0 0 20 20 0 ],[0.95 0.93 0.65 ]);
      | plot([0 60 60 0 0 ],[0 0 20 20 0 ]);
      | patch([25.55 28.44 30.44 32.44 34.44 30.44 27.55 25.55 ],[12.22 12.22 14.22 12.22 14.22 14.22 14.22 12.22 ],[1 1 1 ]);
      | patch([27.55 30.44 28.44 25.55 27.55 ],[10.22 10.22 12.22 12.22 10.22 ],[0.985 0.979 0.895 ]);
      | patch([25.55 28.44 30.44 27.55 25.55 ],[8.22 8.22 10.22 10.22 8.22 ],[1 1 1 ]);
      | patch([27.55 34.44 32.44 30.44 28.44 25.55 27.55 ],[6.22 6.22 8.22 6.22 8.22 8.22 6.22 ],[0.985 0.979 0.895 ]);
      | fprintf('','COMMENT: end icon graphics');
      | fprintf('','COMMENT: begin icon text');
      | color('black');port_label('input',1,' ');
      | color('black');port_label('output',1,'\fontsize{11pt}\bf Out ','texmode','on');
      | fprintf('','COMMENT: end icon text');
      mask prompts: infoedit ""; inherit_from_input_sgadvanced ""; inherit_from_input "Propagate data type to output"; hdl_port_sgadvanced ""; hdl_port "Translate into output port"; timing_constraint_sgadvanced ""; timing_constraint "IOB timing constraint"; locs_specified_sgadvanced ""; locs_specified "Specify IOB location constraints"; LOCs "IOB pad locations (cell array {'MSB', ..., 'LSB'})"; xl_use_area_sgadvanced ""; xl_use_area "Define FPGA area for resource estimation"; xl_area "FPGA area [slices, FFs, BRAMs, LUTs, IOBs, emb. mults, TBUFs]"; UseAsDAC_sgadvanced ""; UseAsDAC "Drive DAC Input"; DACChannel "DAC Channel ID"; sginterface ""; has_advanced_control ""; sggui_pos ""; block_type ""; block_version ""; sg_icon_stat ""; sg_mask_display ""; sg_list_contents ""; sg_blockgui_xml ""
      mask help:
      | Gateway out block.  Converts Xilinx fixed-point or floating-point type inputs into ouputs of type Simulink integer, single, double, or fixed point.
      |
      | Hardware notes:  In hardware these blocks become top level output ports or are discarded, depending on how they are configured.
      mask init:
      | try
      |   tmp_gcb = gcb;
      |   tmp_gcbh = gcbh;
      |   if (strcmp('SysGenIndex',get_param(bdroot(tmp_gcbh),'tag')) && ~isempty(regexp(bdroot(tmp_gcb), '^xbs', 'once')))
      |     return;
      |   end;
      |   xlMungeMaskParams;
      |   block_config = 'sysgen_blockset:gateway_out_config';
      | 
      |   block_type='gatewayout';
      | 
      |   serialized_declarations = '{''DACChannel''=>''String'',''LOCs''=>''StringVector'',''UseAsDAC''=>''Int'',''hdl_port''=>''Int'',''inherit_from_input''=>''Int'',''locs_specified''=>''Int'',''sginterface''=>''String'',''timing_constraint''=>''Int'',''block_type''=>''String''}';
      |   ptable_ = xlblockprep(get_param(tmp_gcb, 'MaskWSVariables'));
      |   try
      |     xlBlockMoveCallback(tmp_gcbh);
      |   catch 
      |      clear global xl_updateicon_recursion_guard;
      |   end;
      | catch
      |   global dbgsysgen;
      |   if(~isempty(dbgsysgen) && dbgsysgen)
      |     e = regexprep(lasterr, '\n', '\nError: ');
      |     disp(['Error: While running MaskInit code on block ' tmp_gcb ': ' e]);
      |     error(e);
      |   end
      | end
      settings: CopyFcn=xlBlockMoveCallback(gcbh);  DeleteFcn=xlDestroyGui(gcbh);  ModelCloseFcn=xlDestroyGui(gcbh);  PreSaveFcn=xlBlockPreSaveCallback(gcbh);  PostSaveFcn=xlBlockPostSaveCallback(gcbh);  DestroyFcn=xlDestroyGui(gcbh);  OpenFcn=xlOpenGui(gcbh, 'gatewayout_gui.xml', @gatewayoutenablement, -1)  CloseFcn=xlDestroyGui(gcbh);  MoveFcn=xlBlockMoveCallback(gcbh);
      mask Help: eval('');xlDoc('-book','sysgen','-topic','Gateway_Out');
      mask StyleString: edit,edit,checkbox,edit,checkbox,edit,popup(None|Data Rate|Data Rate;  Set 'FAST' Attribute),edit,checkbox,edit,edit,checkbox,edit,edit,checkbox,edit,edit,edit,edit,edit,edit,edit,edit,edit,edit
      mask Display:
      | fprintf('','COMMENT: begin icon graphics');
      | patch([0 60 60 0 0 ],[0 0 20 20 0 ],[0.95 0.93 0.65 ]);
      | plot([0 60 60 0 0 ],[0 0 20 20 0 ]);
      | patch([25.55 28.44 30.44 32.44 34.44 30.44 27.55 25.55 ],[12.22 12.22 14.22 12.22 14.22 14.22 14.22 12.22 ],[1 1 1 ]);
      | patch([27.55 30.44 28.44 25.55 27.55 ],[10.22 10.22 12.22 12.22 10.22 ],[0.985 0.979 0.895 ]);
      | patch([25.55 28.44 30.44 27.55 25.55 ],[8.22 8.22 10.22 10.22 8.22 ],[1 1 1 ]);
      | patch([27.55 34.44 32.44 30.44 28.44 25.55 27.55 ],[6.22 6.22 8.22 6.22 8.22 8.22 6.22 ],[0.985 0.979 0.895 ]);
      | fprintf('','COMMENT: end icon graphics');
      | fprintf('','COMMENT: begin icon text');
      | color('black');port_label('input',1,' ');
      | color('black');port_label('output',1,'\fontsize{11pt}\bf Out ','texmode','on');
      | fprintf('','COMMENT: end icon text');
  Indeterminate Probe : Subsystem  LoadFcn=xlBlockLoadCallback(gcbh);  mask(Xilinx Indeterminate Probe Block){infoedit=Produces an output 1 of type double when input data is indeterminate. Output is 0 otherwise.<br><br>Hardware notes: This block and any downstream blocks will be trimmed when hardware is generated., has_advanced_control=0, sggui_pos=-1,-1,-1,-1, block_type=indetprobe, block_version=, sg_icon_stat=25,26,-1,-1,white,yellow,4,07734,right,,[ ],[ ], sg_mask_display=|, sg_list_contents=, sg_blockgui_xml=}
      mask sg_mask_display=|
      | fprintf('','COMMENT: begin icon graphics');
      | patch([25 24.7598 24.0485 22.8934 21.3388 19.4446 17.2835 14.9386 12.5 10.0614 7.71646 5.55537 3.66117 2.10663 0.951506 0.240184 0 0.240184 0.951506 2.10663 3.66117 5.55537 7.71646 10.0614 12.5 14.9386 17.2835 19.4446 21.3388 22.8934 24.0485 24.7598 25 25 ],[13 15.5362 17.9749 20.2224 22.1924 23.8091 25.0104 25.7502 26 25.7502 25.0104 23.8091 22.1924 20.2224 17.9749 15.5362 13 10.4638 8.02512 5.77759 3.80761 2.1909 0.989566 0.249791 0 0.249791 0.989566 2.1909 3.80761 5.77759 8.02512 10.4638 13 13 ],[0.95 0.93 0.65 ]);
      | plot([25 24.7598 24.0485 22.8934 21.3388 19.4446 17.2835 14.9386 12.5 10.0614 7.71646 5.55537 3.66117 2.10663 0.951506 0.240184 0 0.240184 0.951506 2.10663 3.66117 5.55537 7.71646 10.0614 12.5 14.9386 17.2835 19.4446 21.3388 22.8934 24.0485 24.7598 25 25 ],[13 15.5362 17.9749 20.2224 22.1924 23.8091 25.0104 25.7502 26 25.7502 25.0104 23.8091 22.1924 20.2224 17.9749 15.5362 13 10.4638 8.02512 5.77759 3.80761 2.1909 0.989566 0.249791 0 0.249791 0.989566 2.1909 3.80761 5.77759 8.02512 10.4638 13 13 ]);
      | patch([5.325 9.66 12.66 15.66 18.66 12.66 8.325 5.325 ],[16.33 16.33 19.33 16.33 19.33 19.33 19.33 16.33 ],[1 1 1 ]);
      | patch([8.325 12.66 9.66 5.325 8.325 ],[13.33 13.33 16.33 16.33 13.33 ],[0.985 0.979 0.895 ]);
      | patch([5.325 9.66 12.66 8.325 5.325 ],[10.33 10.33 13.33 13.33 10.33 ],[1 1 1 ]);
      | patch([8.325 18.66 15.66 12.66 9.66 5.325 8.325 ],[7.33 7.33 10.33 7.33 10.33 10.33 7.33 ],[0.985 0.979 0.895 ]);
      | fprintf('','COMMENT: end icon graphics');
      | fprintf('','COMMENT: begin icon text');
      | fprintf('','COMMENT: end icon text');disp('!def');
      mask prompts: infoedit ""; has_advanced_control ""; sggui_pos ""; block_type ""; block_version ""; sg_icon_stat ""; sg_mask_display ""; sg_list_contents ""; sg_blockgui_xml ""
      mask help:
      | Produces an output 1 of type double when input data is indeterminate. Output is 0 otherwise.
      |
      | Hardware notes: This block and any downstream blocks will be trimmed when hardware is generated.
      mask init:
      | try
      |   tmp_gcb = gcb;
      |   tmp_gcbh = gcbh;
      |   if (strcmp('SysGenIndex',get_param(bdroot(tmp_gcbh),'tag')) && ~isempty(regexp(bdroot(tmp_gcb), '^xbs', 'once')))
      |     return;
      |   end;
      |   xlMungeMaskParams;
      | 
      |   block_type='indetprobe';
      | 
      |   serialized_declarations = '{''block_type''=>''String''}';
      |   xlindetprobe_init();
      |   ptable_ = xlblockprep(get_param(tmp_gcb, 'MaskWSVariables'));
      |   try
      |     xlBlockMoveCallback(tmp_gcbh);
      |   catch 
      |      clear global xl_updateicon_recursion_guard;
      |   end;
      | catch
      |   global dbgsysgen;
      |   if(~isempty(dbgsysgen) && dbgsysgen)
      |     e = regexprep(lasterr, '\n', '\nError: ');
      |     disp(['Error: While running MaskInit code on block ' tmp_gcb ': ' e]);
      |     error(e);
      |   end
      | end
      settings: CopyFcn=xlBlockMoveCallback(gcbh);  DeleteFcn=xlDestroyGui(gcbh);  ModelCloseFcn=xlDestroyGui(gcbh);  PreSaveFcn=xlBlockPreSaveCallback(gcbh);  PostSaveFcn=xlBlockPostSaveCallback(gcbh);  DestroyFcn=xlDestroyGui(gcbh);  OpenFcn=xlOpenGui(gcbh, 'indetprobe_gui.xml', -1, -1)  CloseFcn=xlDestroyGui(gcbh);  MoveFcn=xlBlockMoveCallback(gcbh);
      mask Help: eval('');xlDoc('-book','sysgen','-topic','Indeterminate_Probe');
      mask Display:
      | fprintf('','COMMENT: begin icon graphics');
      | patch([25 24.7598 24.0485 22.8934 21.3388 19.4446 17.2835 14.9386 12.5 10.0614 7.71646 5.55537 3.66117 2.10663 0.951506 0.240184 0 0.240184 0.951506 2.10663 3.66117 5.55537 7.71646 10.0614 12.5 14.9386 17.2835 19.4446 21.3388 22.8934 24.0485 24.7598 25 25 ],[13 15.5362 17.9749 20.2224 22.1924 23.8091 25.0104 25.7502 26 25.7502 25.0104 23.8091 22.1924 20.2224 17.9749 15.5362 13 10.4638 8.02512 5.77759 3.80761 2.1909 0.989566 0.249791 0 0.249791 0.989566 2.1909 3.80761 5.77759 8.02512 10.4638 13 13 ],[0.95 0.93 0.65 ]);
      | plot([25 24.7598 24.0485 22.8934 21.3388 19.4446 17.2835 14.9386 12.5 10.0614 7.71646 5.55537 3.66117 2.10663 0.951506 0.240184 0 0.240184 0.951506 2.10663 3.66117 5.55537 7.71646 10.0614 12.5 14.9386 17.2835 19.4446 21.3388 22.8934 24.0485 24.7598 25 25 ],[13 15.5362 17.9749 20.2224 22.1924 23.8091 25.0104 25.7502 26 25.7502 25.0104 23.8091 22.1924 20.2224 17.9749 15.5362 13 10.4638 8.02512 5.77759 3.80761 2.1909 0.989566 0.249791 0 0.249791 0.989566 2.1909 3.80761 5.77759 8.02512 10.4638 13 13 ]);
      | patch([5.325 9.66 12.66 15.66 18.66 12.66 8.325 5.325 ],[16.33 16.33 19.33 16.33 19.33 19.33 19.33 16.33 ],[1 1 1 ]);
      | patch([8.325 12.66 9.66 5.325 8.325 ],[13.33 13.33 16.33 16.33 13.33 ],[0.985 0.979 0.895 ]);
      | patch([5.325 9.66 12.66 8.325 5.325 ],[10.33 10.33 13.33 13.33 10.33 ],[1 1 1 ]);
      | patch([8.325 18.66 15.66 12.66 9.66 5.325 8.325 ],[7.33 7.33 10.33 7.33 10.33 10.33 7.33 ],[0.985 0.979 0.895 ]);
      | fprintf('','COMMENT: end icon graphics');
      | fprintf('','COMMENT: begin icon text');
      | fprintf('','COMMENT: end icon text');disp('!def');
  "Interleaver Deinterleaver 5.1 " : S-Function  LoadFcn=xlBlockLoadCallback(gcbh);  FunctionName=sysgen  Parameters=ptable_  EnableBusSupport=off  mask(Xilinx Interleaver/Deinterleaver 5.1 Block){mode_sgadvanced=, mode=Interleaver, num_branches=3, branch_length=[2 4 5], rst_sgadvanced=, rst=off, en_sgadvanced=, en=off, dbl_ovrd_sgadvanced=, dbl_ovrd=off, explicit_period_sgadvanced=, explicit_period=off, period=1, mem_type_sgadvanced=, mem_type=Automatically Chosen, pipeline_sgadvanced=, pipeline=off, use_rpm_sgadvanced=, use_rpm=on, xl_use_area_sgadvanced=, xl_use_area=off, xl_area=[0,0,0,0,0,0,0], useCore=, version=51, has_advanced_control=0, sggui_pos=-1,-1,-1,-1, block_type=interleaver_deinterleaver_v5_1, block_version=, sg_icon_stat=60,58,2,2,white,green,0,843f4b9c,right,,[ ],[ ], sg_mask_display=|, sg_list_contents=, sg_blockgui_xml=}
      mask sg_mask_display=|
      | fprintf('','COMMENT: begin icon graphics');
      | patch([0 60 60 0 0 ],[0 0 58 58 0 ],[0.72 0.84 0.7 ]);
      | plot([0 60 60 0 0 ],[0 0 58 58 0 ]);
      | patch([12.2 23.76 31.76 39.76 47.76 31.76 20.2 12.2 ],[37.88 37.88 45.88 37.88 45.88 45.88 45.88 37.88 ],[1 1 1 ]);
      | patch([20.2 31.76 23.76 12.2 20.2 ],[29.88 29.88 37.88 37.88 29.88 ],[0.916 0.952 0.91 ]);
      | patch([12.2 23.76 31.76 20.2 12.2 ],[21.88 21.88 29.88 29.88 21.88 ],[1 1 1 ]);
      | patch([20.2 47.76 39.76 31.76 23.76 12.2 20.2 ],[13.88 13.88 21.88 13.88 21.88 21.88 13.88 ],[0.916 0.952 0.91 ]);
      | fprintf('','COMMENT: end icon graphics');
      | fprintf('','COMMENT: begin icon text');
      | color('black');port_label('input',1,'din');
      | color('black');port_label('input',2,'vin');
      | color('black');port_label('output',1,'dout');
      | color('black');port_label('output',2,'vout');
      | fprintf('','COMMENT: end icon text');
      mask prompts: mode_sgadvanced ""; num_branches "Number of branches"; branch_length "Lengths of branches"; rst_sgadvanced ""; rst "Provide synchronous reset port"; en_sgadvanced ""; en "Provide enable port"; dbl_ovrd_sgadvanced ""; dbl_ovrd "Override with doubles"; explicit_period_sgadvanced ""; explicit_period "Specify explicit sample period"; period ""; mem_type_sgadvanced ""; mem_type "Memory type"; pipeline_sgadvanced ""; pipeline "Pipeline for maximum performance"; use_rpm_sgadvanced ""; use_rpm "Use core placement information"; xl_use_area_sgadvanced ""; xl_use_area "Define FPGA area for resource estimation"; xl_area "FPGA area [slices, FFs, BRAMs, LUTs, IOBs, emb. mults, TBUFs]"; useCore ""; version ""; has_advanced_control ""; sggui_pos ""; block_type ""; block_version ""; sg_icon_stat ""; sg_mask_display ""; sg_list_contents ""; sg_blockgui_xml ""
      mask help: Xilinx Interleaver/Deinterleaver 5.1
      mask init:
      | try
      |   tmp_gcb = gcb;
      |   tmp_gcbh = gcbh;
      |   if (strcmp('SysGenIndex',get_param(bdroot(tmp_gcbh),'tag')) && ~isempty(regexp(bdroot(tmp_gcb), '^xbs', 'once')))
      |     return;
      |   end;
      |   xlMungeMaskParams;
      |   block_config = 'sysgen_blockset:Interleaver_config';
      | 
      |   block_type='interleaver_deinterleaver_v5_1';
      | 
      |   serialized_declarations = '{''branch_length''=>''IntVector'',''dbl_ovrd''=>''Bool'',''en''=>''Bool'',''explicit_period''=>''Bool'',''mem_type''=>''Int'',''mode''=>''Int'',''num_branches''=>''Int'',''period''=>''Double'',''pipeline''=>''Bool'',''rst''=>''Bool'',''use_rpm''=>''Bool'',''version''=>''Int'',''block_type''=>''String''}';
      |   ptable_ = xlblockprep(get_param(tmp_gcb, 'MaskWSVariables'));
      |   try
      |     xlBlockMoveCallback(tmp_gcbh);
      |   catch 
      |      clear global xl_updateicon_recursion_guard;
      |   end;
      | catch
      |   global dbgsysgen;
      |   if(~isempty(dbgsysgen) && dbgsysgen)
      |     e = regexprep(lasterr, '\n', '\nError: ');
      |     disp(['Error: While running MaskInit code on block ' tmp_gcb ': ' e]);
      |     error(e);
      |   end
      | end
      settings: CopyFcn=xlBlockMoveCallback(gcbh);  DeleteFcn=xlDestroyGui(gcbh);  ModelCloseFcn=xlDestroyGui(gcbh);  PreSaveFcn=xlBlockPreSaveCallback(gcbh);  PostSaveFcn=xlBlockPostSaveCallback(gcbh);  DestroyFcn=xlDestroyGui(gcbh);  OpenFcn=xlOpenGui(gcbh, 'interleaverv51_gui.xml', @xlmagicenablement, -1)  CloseFcn=xlDestroyGui(gcbh);  MoveFcn=xlBlockMoveCallback(gcbh);
      mask Help: eval('');xlDoc('-book','sysgen','-topic','Interleaver_Deinterleaver_5_1');
      mask StyleString: edit,popup(Interleaver|Deinterleaver),edit,edit,edit,checkbox,edit,checkbox,edit,checkbox,edit,checkbox,edit,edit,popup(Automatically Chosen|Block RAM|Distributed RAM),edit,checkbox,edit,checkbox,edit,checkbox,edit,edit,edit,edit,edit,edit,edit,edit,edit,edit,edit
      mask Display:
      | fprintf('','COMMENT: begin icon graphics');
      | patch([0 60 60 0 0 ],[0 0 58 58 0 ],[0.72 0.84 0.7 ]);
      | plot([0 60 60 0 0 ],[0 0 58 58 0 ]);
      | patch([12.2 23.76 31.76 39.76 47.76 31.76 20.2 12.2 ],[37.88 37.88 45.88 37.88 45.88 45.88 45.88 37.88 ],[1 1 1 ]);
      | patch([20.2 31.76 23.76 12.2 20.2 ],[29.88 29.88 37.88 37.88 29.88 ],[0.916 0.952 0.91 ]);
      | patch([12.2 23.76 31.76 20.2 12.2 ],[21.88 21.88 29.88 29.88 21.88 ],[1 1 1 ]);
      | patch([20.2 47.76 39.76 31.76 23.76 12.2 20.2 ],[13.88 13.88 21.88 13.88 21.88 21.88 13.88 ],[0.916 0.952 0.91 ]);
      | fprintf('','COMMENT: end icon graphics');
      | fprintf('','COMMENT: begin icon text');
      | color('black');port_label('input',1,'din');
      | color('black');port_label('input',2,'vin');
      | color('black');port_label('output',1,'dout');
      | color('black');port_label('output',2,'vout');
      | fprintf('','COMMENT: end icon text');
  "Interleaver Deinterleaver v4_0 " : S-Function  LoadFcn=xlBlockLoadCallback(gcbh);  FunctionName=sysgen  Parameters=ptable_  EnableBusSupport=off  mask(Xilinx Interleaver/Deinterleaver Block){mode_sgadvanced=, mode=Interleaver, num_branches=3, branch_length=[2 4 5], rst_sgadvanced=, rst=off, en_sgadvanced=, en=off, dbl_ovrd_sgadvanced=, dbl_ovrd=off, explicit_period_sgadvanced=, explicit_period=off, period=1, mem_type_sgadvanced=, mem_type=Automatically Chosen, pipeline_sgadvanced=, pipeline=off, use_rpm_sgadvanced=, use_rpm=on, xl_use_area_sgadvanced=, xl_use_area=off, xl_area=[0,0,0,0,0,0,0], useCore=, version=4, has_advanced_control=0, sggui_pos=-1,-1,-1,-1, block_type=interleaver_deinterleaver_v4_0, block_version=, sg_icon_stat=60,58,-1,-1,white,green,0,07734,right,,[ ],[ ], sg_mask_display=|, sg_list_contents=, sg_blockgui_xml=}
      mask sg_mask_display=|
      | fprintf('','COMMENT: begin icon graphics');
      | patch([0 60 60 0 0 ],[0 0 58 58 0 ],[0.72 0.84 0.7 ]);
      | plot([0 60 60 0 0 ],[0 0 58 58 0 ]);
      | patch([12.2 23.76 31.76 39.76 47.76 31.76 20.2 12.2 ],[37.88 37.88 45.88 37.88 45.88 45.88 45.88 37.88 ],[1 1 1 ]);
      | patch([20.2 31.76 23.76 12.2 20.2 ],[29.88 29.88 37.88 37.88 29.88 ],[0.916 0.952 0.91 ]);
      | patch([12.2 23.76 31.76 20.2 12.2 ],[21.88 21.88 29.88 29.88 21.88 ],[1 1 1 ]);
      | patch([20.2 47.76 39.76 31.76 23.76 12.2 20.2 ],[13.88 13.88 21.88 13.88 21.88 21.88 13.88 ],[0.916 0.952 0.91 ]);
      | fprintf('','COMMENT: end icon graphics');
      | fprintf('','COMMENT: begin icon text');
      | fprintf('','COMMENT: end icon text');
      mask prompts: mode_sgadvanced ""; num_branches "Number of branches"; branch_length "Lengths of branches"; rst_sgadvanced ""; rst "Provide synchronous reset port"; en_sgadvanced ""; en "Provide enable port"; dbl_ovrd_sgadvanced ""; dbl_ovrd "Override with doubles"; explicit_period_sgadvanced ""; explicit_period "Specify explicit sample period"; period ""; mem_type_sgadvanced ""; mem_type "Memory type"; pipeline_sgadvanced ""; pipeline "Pipeline for maximum performance"; use_rpm_sgadvanced ""; use_rpm "Use core placement information"; xl_use_area_sgadvanced ""; xl_use_area "Define FPGA area for resource estimation"; xl_area "FPGA area [slices, FFs, BRAMs, LUTs, IOBs, emb. mults, TBUFs]"; useCore ""; version ""; has_advanced_control ""; sggui_pos ""; block_type ""; block_version ""; sg_icon_stat ""; sg_mask_display ""; sg_list_contents ""; sg_blockgui_xml ""
      mask help: Xilinx Interleaver/Deinterleaver
      mask init:
      | try
      |   tmp_gcb = gcb;
      |   tmp_gcbh = gcbh;
      |   if (strcmp('SysGenIndex',get_param(bdroot(tmp_gcbh),'tag')) && ~isempty(regexp(bdroot(tmp_gcb), '^xbs', 'once')))
      |     return;
      |   end;
      |   xlMungeMaskParams;
      |   block_config = 'sysgen_blockset:Removed_config';
      | 
      |   block_type='interleaver_deinterleaver_v4_0';
      | nport = get_param(gcbh, 'ports');
      | nin = nport(1);
      | nout = nport(2);
      | 
      |   serialized_declarations = '{''branch_length''=>''IntVector'',''dbl_ovrd''=>''Bool'',''en''=>''Bool'',''explicit_period''=>''Bool'',''mem_type''=>''Int'',''mode''=>''Int'',''num_branches''=>''Int'',''period''=>''Double'',''pipeline''=>''Bool'',''rst''=>''Bool'',''use_rpm''=>''Bool'',''version''=>''Int'',''block_type''=>''String'',''nin''=>''Double'',''nout''=>''Double''}';
      |   ptable_ = xlblockprep(get_param(tmp_gcb, 'MaskWSVariables'));
      |   try
      |     xlBlockMoveCallback(tmp_gcbh);
      |   catch 
      |      clear global xl_updateicon_recursion_guard;
      |   end;
      | catch
      |   global dbgsysgen;
      |   if(~isempty(dbgsysgen) && dbgsysgen)
      |     e = regexprep(lasterr, '\n', '\nError: ');
      |     disp(['Error: While running MaskInit code on block ' tmp_gcb ': ' e]);
      |     error(e);
      |   end
      | end
      settings: CopyFcn=xlBlockMoveCallback(gcbh);  DeleteFcn=xlDestroyGui(gcbh);  ModelCloseFcn=xlDestroyGui(gcbh);  PreSaveFcn=xlBlockPreSaveCallback(gcbh);  PostSaveFcn=xlBlockPostSaveCallback(gcbh);  DestroyFcn=xlDestroyGui(gcbh);  OpenFcn=xlOpenGui(gcbh, 'interleaver_gui.xml', @xlremovedenablement, -1)  CloseFcn=xlDestroyGui(gcbh);  MoveFcn=xlBlockMoveCallback(gcbh);
      mask Help: eval('');xlDoc('-book','sysgen','-topic','Interleaver_Deinterleaver_v4_0');
      mask StyleString: edit,popup(Interleaver|Deinterleaver),edit,edit,edit,checkbox,edit,checkbox,edit,checkbox,edit,checkbox,edit,edit,popup(Automatically Chosen|Block RAM|Distributed RAM),edit,checkbox,edit,checkbox,edit,checkbox,edit,edit,edit,edit,edit,edit,edit,edit,edit,edit,edit
      mask Display:
      | fprintf('','COMMENT: begin icon graphics');
      | patch([0 60 60 0 0 ],[0 0 58 58 0 ],[0.72 0.84 0.7 ]);
      | plot([0 60 60 0 0 ],[0 0 58 58 0 ]);
      | patch([12.2 23.76 31.76 39.76 47.76 31.76 20.2 12.2 ],[37.88 37.88 45.88 37.88 45.88 45.88 45.88 37.88 ],[1 1 1 ]);
      | patch([20.2 31.76 23.76 12.2 20.2 ],[29.88 29.88 37.88 37.88 29.88 ],[0.916 0.952 0.91 ]);
      | patch([12.2 23.76 31.76 20.2 12.2 ],[21.88 21.88 29.88 29.88 21.88 ],[1 1 1 ]);
      | patch([20.2 47.76 39.76 31.76 23.76 12.2 20.2 ],[13.88 13.88 21.88 13.88 21.88 21.88 13.88 ],[0.916 0.952 0.91 ]);
      | fprintf('','COMMENT: end icon graphics');
      | fprintf('','COMMENT: begin icon text');
      | fprintf('','COMMENT: end icon text');
  "Interleaver Deinterleaver v5_0 " : S-Function  LoadFcn=xlBlockLoadCallback(gcbh);  FunctionName=sysgen  Parameters=ptable_  EnableBusSupport=off  mask(Xilinx Interleaver/Deinterleaver Block){mode_sgadvanced=, mode=Interleaver, num_branches=3, branch_length=[2 4 5], rst_sgadvanced=, rst=off, en_sgadvanced=, en=off, dbl_ovrd_sgadvanced=, dbl_ovrd=off, explicit_period_sgadvanced=, explicit_period=off, period=1, mem_type_sgadvanced=, mem_type=Automatically Chosen, pipeline_sgadvanced=, pipeline=off, use_rpm_sgadvanced=, use_rpm=on, xl_use_area_sgadvanced=, xl_use_area=off, xl_area=[0,0,0,0,0,0,0], useCore=, version=5, has_advanced_control=0, sggui_pos=-1,-1,-1,-1, block_type=interleaver_deinterleaver_v5_0, block_version=, sg_icon_stat=60,58,-1,-1,white,green,0,07734,right,,[ ],[ ], sg_mask_display=|, sg_list_contents=, sg_blockgui_xml=}
      mask sg_mask_display=|
      | fprintf('','COMMENT: begin icon graphics');
      | patch([0 60 60 0 0 ],[0 0 58 58 0 ],[0.72 0.84 0.7 ]);
      | plot([0 60 60 0 0 ],[0 0 58 58 0 ]);
      | patch([12.2 23.76 31.76 39.76 47.76 31.76 20.2 12.2 ],[37.88 37.88 45.88 37.88 45.88 45.88 45.88 37.88 ],[1 1 1 ]);
      | patch([20.2 31.76 23.76 12.2 20.2 ],[29.88 29.88 37.88 37.88 29.88 ],[0.916 0.952 0.91 ]);
      | patch([12.2 23.76 31.76 20.2 12.2 ],[21.88 21.88 29.88 29.88 21.88 ],[1 1 1 ]);
      | patch([20.2 47.76 39.76 31.76 23.76 12.2 20.2 ],[13.88 13.88 21.88 13.88 21.88 21.88 13.88 ],[0.916 0.952 0.91 ]);
      | fprintf('','COMMENT: end icon graphics');
      | fprintf('','COMMENT: begin icon text');
      | fprintf('','COMMENT: end icon text');
      mask prompts: mode_sgadvanced ""; num_branches "Number of branches"; branch_length "Lengths of branches"; rst_sgadvanced ""; rst "Provide synchronous reset port"; en_sgadvanced ""; en "Provide enable port"; dbl_ovrd_sgadvanced ""; dbl_ovrd "Override with doubles"; explicit_period_sgadvanced ""; explicit_period "Specify explicit sample period"; period ""; mem_type_sgadvanced ""; mem_type "Memory type"; pipeline_sgadvanced ""; pipeline "Pipeline for maximum performance"; use_rpm_sgadvanced ""; use_rpm "Use core placement information"; xl_use_area_sgadvanced ""; xl_use_area "Define FPGA area for resource estimation"; xl_area "FPGA area [slices, FFs, BRAMs, LUTs, IOBs, emb. mults, TBUFs]"; useCore ""; version ""; has_advanced_control ""; sggui_pos ""; block_type ""; block_version ""; sg_icon_stat ""; sg_mask_display ""; sg_list_contents ""; sg_blockgui_xml ""
      mask help: Xilinx Interleaver/Deinterleaver
      mask init:
      | try
      |   tmp_gcb = gcb;
      |   tmp_gcbh = gcbh;
      |   if (strcmp('SysGenIndex',get_param(bdroot(tmp_gcbh),'tag')) && ~isempty(regexp(bdroot(tmp_gcb), '^xbs', 'once')))
      |     return;
      |   end;
      |   xlMungeMaskParams;
      |   block_config = 'sysgen_blockset:Removed_config';
      | 
      |   block_type='interleaver_deinterleaver_v5_0';
      | nport = get_param(gcbh, 'ports');
      | nin = nport(1);
      | nout = nport(2);
      | 
      |   serialized_declarations = '{''branch_length''=>''IntVector'',''dbl_ovrd''=>''Bool'',''en''=>''Bool'',''explicit_period''=>''Bool'',''mem_type''=>''Int'',''mode''=>''Int'',''num_branches''=>''Int'',''period''=>''Double'',''pipeline''=>''Bool'',''rst''=>''Bool'',''use_rpm''=>''Bool'',''version''=>''Int'',''block_type''=>''String'',''nin''=>''Double'',''nout''=>''Double''}';
      |   ptable_ = xlblockprep(get_param(tmp_gcb, 'MaskWSVariables'));
      |   try
      |     xlBlockMoveCallback(tmp_gcbh);
      |   catch 
      |      clear global xl_updateicon_recursion_guard;
      |   end;
      | catch
      |   global dbgsysgen;
      |   if(~isempty(dbgsysgen) && dbgsysgen)
      |     e = regexprep(lasterr, '\n', '\nError: ');
      |     disp(['Error: While running MaskInit code on block ' tmp_gcb ': ' e]);
      |     error(e);
      |   end
      | end
      settings: CopyFcn=xlBlockMoveCallback(gcbh);  DeleteFcn=xlDestroyGui(gcbh);  ModelCloseFcn=xlDestroyGui(gcbh);  PreSaveFcn=xlBlockPreSaveCallback(gcbh);  PostSaveFcn=xlBlockPostSaveCallback(gcbh);  DestroyFcn=xlDestroyGui(gcbh);  OpenFcn=xlOpenGui(gcbh, 'interleaverv5_gui.xml', @xlremovedenablement, -1)  CloseFcn=xlDestroyGui(gcbh);  MoveFcn=xlBlockMoveCallback(gcbh);
      mask Help: eval('');xlDoc('-book','sysgen','-topic','Interleaver_Deinterleaver_v5_0');
      mask StyleString: edit,popup(Interleaver|Deinterleaver),edit,edit,edit,checkbox,edit,checkbox,edit,checkbox,edit,checkbox,edit,edit,popup(Automatically Chosen|Block RAM|Distributed RAM),edit,checkbox,edit,checkbox,edit,checkbox,edit,edit,edit,edit,edit,edit,edit,edit,edit,edit,edit
      mask Display:
      | fprintf('','COMMENT: begin icon graphics');
      | patch([0 60 60 0 0 ],[0 0 58 58 0 ],[0.72 0.84 0.7 ]);
      | plot([0 60 60 0 0 ],[0 0 58 58 0 ]);
      | patch([12.2 23.76 31.76 39.76 47.76 31.76 20.2 12.2 ],[37.88 37.88 45.88 37.88 45.88 45.88 45.88 37.88 ],[1 1 1 ]);
      | patch([20.2 31.76 23.76 12.2 20.2 ],[29.88 29.88 37.88 37.88 29.88 ],[0.916 0.952 0.91 ]);
      | patch([12.2 23.76 31.76 20.2 12.2 ],[21.88 21.88 29.88 29.88 21.88 ],[1 1 1 ]);
      | patch([20.2 47.76 39.76 31.76 23.76 12.2 20.2 ],[13.88 13.88 21.88 13.88 21.88 21.88 13.88 ],[0.916 0.952 0.91 ]);
      | fprintf('','COMMENT: end icon graphics');
      | fprintf('','COMMENT: begin icon text');
      | fprintf('','COMMENT: end icon text');
  "Interleaver/De-interleaver 6.0 " : S-Function  LoadFcn=xlBlockLoadCallback(gcbh);  FunctionName=sysgen  Parameters=ptable_  EnableBusSupport=off  mask(Xilinx Interleaver De-interleaver 6.0  Block){infoedit=Forney Information : The Forney type is composed of a user-defined number of delay-line shift registers. The length of each of the delay-line shift registers can be specified using a COE file, or by setting the difference in the length of consecutive delay line shift registers to a fixed, user-defined value. <br> Rectangular Information : The Rectangular Block type is composed of a rectangular array of memory elements, where the number of rows and columns in the array is user-defined. The number of rows and columns can be constant or run-time configurable. The elements are written to row-wise, and read out column-wise, or vice versa, depending on which mode is selected. This type supports user-defined inter-row and inter-column permutations. It also supports pruning - cases where the block size is less than the product of the number of rows and columns., memory_style=automatic, symbol_width=1, sid_type_sgadvanced=, sid_type=forney, mode_sgadvanced=, mode=interleaver, symbol_memory_sgadvanced=, symbol_memory=internal, number_of_branches=16, architecture_sgadvanced=, architecture=rom_based, number_of_configurations=1, branch_length_constant=1, branch_length_coe_file_name='no_coe_file_loaded', branch_length_type_sgadvanced=, branch_length_type=constant_difference_between_consecutive_branches, number_of_rows_constant_value=15, row_port_width=4, minimum_rows=15, number_of_rows_selectable_value=4, number_of_rows_sgadvanced=, number_of_rows=constant, number_of_columns_constant_value=15, col_port_width=2, minimum_columns=2, number_of_columns_selectable_value=4, number_of_columns_sgadvanced=, number_of_columns=constant, row_permutations_sgadvanced=, row_permutations=none, column_permutations_sgadvanced=, column_permutations=none, coe_file='no_coe_file_loaded', block_size_constant_value=225, block_size_port_width=3, block_size_type_sgadvanced=, block_size_type=constant, row_valid_sgadvanced=, row_valid=off, block_size_valid_sgadvanced=, block_size_valid=off, ce_sgadvanced=, ce=off, rfd_sgadvanced=, rfd=off, row_sel_valid_sgadvanced=, row_sel_valid=off, block_start_sgadvanced=, block_start=off, sclr_sgadvanced=, sclr=off, rffd_sgadvanced=, rffd=off, col_valid_sgadvanced=, col_valid=off, block_end_sgadvanced=, block_end=off, ndo_sgadvanced=, ndo=off, fdo_sgadvanced=, fdo=off, col_sel_valid_sgadvanced=, col_sel_valid=off, nd_sgadvanced=, nd=on, rdy_sgadvanced=, rdy=off, pipelining_sgadvanced=, pipelining=minimum, ip_name=Interleaver/De-interleaver, ip_version=6.0, dsptool_ready=true, ipcore_usecache=true, ipcore_useipmodelcache=true, wrapper_available=true, port_translation_map={ 'ce' => 'en', 'sclr' => 'rst'}, structural_sim=false, ipcore_verbose=false, ipcore_do_not_force_period=true, has_advanced_control=0, sggui_pos=-1,-1,-1,-1, block_type=sid_v6_0, block_version=, sg_icon_stat=95,142,3,1,white,green,0,e6536295,right,,[ ],[ ], sg_mask_display=|, sg_list_contents=, sg_blockgui_xml=}
      mask sg_mask_display=|
      | fprintf('','COMMENT: begin icon graphics');
      | patch([0 95 95 0 0 ],[0 0 142 142 0 ],[0.72 0.84 0.7 ]);
      | plot([0 95 95 0 0 ],[0 0 142 142 0 ]);
      | patch([18.075 36.86 49.86 62.86 75.86 49.86 31.075 18.075 ],[85.43 85.43 98.43 85.43 98.43 98.43 98.43 85.43 ],[1 1 1 ]);
      | patch([31.075 49.86 36.86 18.075 31.075 ],[72.43 72.43 85.43 85.43 72.43 ],[0.916 0.952 0.91 ]);
      | patch([18.075 36.86 49.86 31.075 18.075 ],[59.43 59.43 72.43 72.43 59.43 ],[1 1 1 ]);
      | patch([31.075 75.86 62.86 49.86 36.86 18.075 31.075 ],[46.43 46.43 59.43 46.43 59.43 59.43 46.43 ],[0.916 0.952 0.91 ]);
      | fprintf('','COMMENT: end icon graphics');
      | fprintf('','COMMENT: begin icon text');
      | color('black');port_label('input',1,'din');
      | color('black');port_label('input',2,'nd');
      | color('black');port_label('input',3,'fd');
      | color('black');port_label('output',1,'dout');
      | fprintf('','COMMENT: end icon text');
      mask prompts: infoedit ""; memory_style "Memory Style"; symbol_width "Symbol Width"; sid_type_sgadvanced ""; sid_type ""; mode_sgadvanced ""; mode ""; symbol_memory_sgadvanced ""; symbol_memory ""; number_of_branches "Number of branches"; architecture_sgadvanced ""; architecture ""; number_of_configurations "Number of configurations"; branch_length_constant "Value"; branch_length_coe_file_name "COE File"; branch_length_type_sgadvanced ""; branch_length_type "Branch length descriptions for Forney SID."; number_of_rows_constant_value "Value"; row_port_width "Row Port Width"; minimum_rows "Minimum Number of Rows"; number_of_rows_selectable_value "Number of Values"; number_of_rows_sgadvanced ""; number_of_rows ""; number_of_columns_constant_value "Value"; col_port_width "COL Port Width"; minimum_columns "Minimum Number of Columns"; number_of_columns_selectable_value "Number of Values"; number_of_columns_sgadvanced ""; number_of_columns ""; row_permutations_sgadvanced ""; row_permutations "Row permutation"; column_permutations_sgadvanced ""; column_permutations "Column permutations"; coe_file "COE File"; block_size_constant_value "Value"; block_size_port_width "BLOCK_SIZE Port Width"; block_size_type_sgadvanced ""; block_size_type ""; row_valid_sgadvanced ""; block_size_valid_sgadvanced ""; ce_sgadvanced ""; rfd_sgadvanced ""; row_sel_valid_sgadvanced ""; block_start_sgadvanced ""; sclr_sgadvanced ""; rffd_sgadvanced ""; col_valid_sgadvanced ""; block_end_sgadvanced ""; ndo_sgadvanced ""; fdo_sgadvanced ""; col_sel_valid_sgadvanced ""; nd_sgadvanced ""; rdy_sgadvanced ""; pipelining_sgadvanced ""; pipelining ""; ip_name ""; ip_version ""; dsptool_ready ""; ipcore_usecache ""; ipcore_useipmodelcache ""; wrapper_available ""; port_translation_map ""; structural_sim ""; ipcore_verbose ""; ipcore_do_not_force_period ""; has_advanced_control ""; sggui_pos ""; block_type ""; block_version ""; sg_icon_stat ""; sg_mask_display ""; sg_list_contents ""; sg_blockgui_xml ""
      mask help:
      | Forney Information : The Forney type is composed of a user-defined number of delay-line shift registers. The length of each of the delay-line shift registers can be specified using a COE file, or by setting the difference in the length of consecutive delay line shift registers to a fixed, user-defined value.
      |  Rectangular Information : The Rectangular Block type is composed of a rectangular array of memory elements, where the number of rows and columns in the array is user-defined. The number of rows and columns can be constant or run-time configurable. The elements are written to row-wise, and read out column-wise, or vice versa, depending on which mode is selected. This type supports user-defined inter-row and inter-column permutations. It also supports pruning - cases where the block size is less than the product of the number of rows and columns.
      mask init:
      | try
      |   tmp_gcb = gcb;
      |   tmp_gcbh = gcbh;
      |   if (strcmp('SysGenIndex',get_param(bdroot(tmp_gcbh),'tag')) && ~isempty(regexp(bdroot(tmp_gcb), '^xbs', 'once')))
      |     return;
      |   end;
      |   xlMungeMaskParams;
      |   block_config = 'sysgen:coregenimport_config';
      | 
      |   block_type='sid_v6_0';
      | 
      |   serialized_declarations = '{''architecture''=>''String'',''block_end''=>''Bool'',''block_size_constant_value''=>''Int'',''block_size_port_width''=>''Int'',''block_size_type''=>''String'',''block_size_valid''=>''Bool'',''block_start''=>''Bool'',''branch_length_coe_file_name''=>''String'',''branch_length_constant''=>''Int'',''branch_length_type''=>''String'',''ce''=>''Bool'',''coe_file''=>''String'',''col_port_width''=>''Int'',''col_sel_valid''=>''Bool'',''col_valid''=>''Bool'',''column_permutations''=>''String'',''dsptool_ready''=>''Bool'',''fdo''=>''Bool'',''ip_name''=>''String'',''ip_version''=>''String'',''ipcore_do_not_force_period''=>''Bool'',''ipcore_usecache''=>''Bool'',''ipcore_useipmodelcache''=>''Bool'',''ipcore_verbose''=>''Bool'',''memory_style''=>''String'',''minimum_columns''=>''Int'',''minimum_rows''=>''Int'',''mode''=>''String'',''nd''=>''Bool'',''ndo''=>''Bool'',''number_of_branches''=>''Int'',''number_of_columns''=>''String'',''number_of_columns_constant_value''=>''Int'',''number_of_columns_selectable_value''=>''Int'',''number_of_configurations''=>''Int'',''number_of_rows''=>''String'',''number_of_rows_constant_value''=>''Int'',''number_of_rows_selectable_value''=>''Int'',''pipelining''=>''String'',''port_translation_map''=>''String'',''rdy''=>''Bool'',''rfd''=>''Bool'',''rffd''=>''Bool'',''row_permutations''=>''String'',''row_port_width''=>''Int'',''row_sel_valid''=>''Bool'',''row_valid''=>''Bool'',''sclr''=>''Bool'',''sid_type''=>''String'',''structural_sim''=>''Bool'',''symbol_memory''=>''String'',''symbol_width''=>''Int'',''wrapper_available''=>''Bool'',''block_type''=>''String''}';
      |   ptable_ = xlblockprep(get_param(tmp_gcb, 'MaskWSVariables'));
      |   try
      |     xlBlockMoveCallback(tmp_gcbh);
      |   catch 
      |      clear global xl_updateicon_recursion_guard;
      |   end;
      | catch
      |   global dbgsysgen;
      |   if(~isempty(dbgsysgen) && dbgsysgen)
      |     e = regexprep(lasterr, '\n', '\nError: ');
      |     disp(['Error: While running MaskInit code on block ' tmp_gcb ': ' e]);
      |     error(e);
      |   end
      | end
      settings: CopyFcn=xlBlockMoveCallback(gcbh);  DeleteFcn=xlDestroyGui(gcbh);  ModelCloseFcn=xlDestroyGui(gcbh);  PreSaveFcn=xlBlockPreSaveCallback(gcbh);  PostSaveFcn=xlBlockPostSaveCallback(gcbh);  DestroyFcn=xlDestroyGui(gcbh);  OpenFcn=xlOpenGui(gcbh, 'sid_v6_0_gui.xml', @sid_v6_0_enablement, @sid_v6_0_action)  CloseFcn=xlDestroyGui(gcbh);  MoveFcn=xlBlockMoveCallback(gcbh);
      mask Help: eval('');xlDoc('-book','sysgen','-topic','Interleaver__De_interleaver_6_0');
      mask StyleString: edit,popup(automatic|block|distributed),edit,edit,popup(forney|rectangular),edit,popup(interleaver|deinterleaver),edit,popup(internal|external),edit,edit,popup(rom_based|logic_based),edit,edit,edit,edit,popup(constant_difference_between_consecutive_branches|use_coe_file_to_define_branch_lengths|coe_file_defines_individual_branch_lengths_for_every_branch_in_each_configuration|coe_file_defines_branch_length_constant_for_each_configuration),edit,edit,edit,edit,edit,popup(constant|variable|selectable),edit,edit,edit,edit,edit,popup(constant|variable|selectable),edit,popup(none|use_coe_file_to_define_row_permutations),edit,popup(none|use_coe_file_to_define_column_permutations),edit,edit,edit,edit,popup(constant|rows_columns|variable),edit,checkbox,edit,checkbox,edit,checkbox,edit,checkbox,edit,checkbox,edit,checkbox,edit,checkbox,edit,checkbox,edit,checkbox,edit,checkbox,edit,checkbox,edit,checkbox,edit,checkbox,edit,checkbox,edit,checkbox,edit,popup(minimum|medium|maximum),edit,edit,edit,edit,edit,edit,edit,edit,edit,edit,edit,edit,edit,edit,edit,edit,edit,edit
      mask Display:
      | fprintf('','COMMENT: begin icon graphics');
      | patch([0 95 95 0 0 ],[0 0 142 142 0 ],[0.72 0.84 0.7 ]);
      | plot([0 95 95 0 0 ],[0 0 142 142 0 ]);
      | patch([18.075 36.86 49.86 62.86 75.86 49.86 31.075 18.075 ],[85.43 85.43 98.43 85.43 98.43 98.43 98.43 85.43 ],[1 1 1 ]);
      | patch([31.075 49.86 36.86 18.075 31.075 ],[72.43 72.43 85.43 85.43 72.43 ],[0.916 0.952 0.91 ]);
      | patch([18.075 36.86 49.86 31.075 18.075 ],[59.43 59.43 72.43 72.43 59.43 ],[1 1 1 ]);
      | patch([31.075 75.86 62.86 49.86 36.86 18.075 31.075 ],[46.43 46.43 59.43 46.43 59.43 59.43 46.43 ],[0.916 0.952 0.91 ]);
      | fprintf('','COMMENT: end icon graphics');
      | fprintf('','COMMENT: begin icon text');
      | color('black');port_label('input',1,'din');
      | color('black');port_label('input',2,'nd');
      | color('black');port_label('input',3,'fd');
      | color('black');port_label('output',1,'dout');
      | fprintf('','COMMENT: end icon text');
  "Interleaver/De-interleaver 7.0 " : S-Function  LoadFcn=xlBlockLoadCallback(gcbh);  FunctionName=sysgen  Parameters=ptable_  EnableBusSupport=off  mask(Xilinx Interleaver De-interleaver 7.0  Block){infoedit=Forney Information : The Forney type is composed of a user-defined number of delay-line shift registers. The length of each of the delay-line shift registers can be specified using a COE file, or by setting the difference in the length of consecutive delay line shift registers to a fixed, user-defined value. <br> Rectangular Information : The Rectangular Block type is composed of a rectangular array of memory elements, where the number of rows and columns in the array is user-defined. The number of rows and columns can be constant or run-time configurable. The elements are written to row-wise, and read out column-wise, or vice versa, depending on which mode is selected. This type supports user-defined inter-row and inter-column permutations. It also supports pruning - cases where the block size is less than the product of the number of rows and columns., memory_style=automatic, symbol_width=1, sid_type_sgadvanced=, sid_type=forney, mode_sgadvanced=, mode=interleaver, external_memory_latency=0, symbol_memory_sgadvanced=, symbol_memory=internal, number_of_branches=16, architecture_sgadvanced=, architecture=rom_based, number_of_configurations=1, branch_length_type_sgadvanced=, branch_length_type=constant_difference_between_consecutive_branches, branch_length_constant=1, branch_length_coe_file_name='no_coe_file_loaded', number_of_rows_constant_value=15, row_port_width=4, minimum_rows=15, number_of_rows_selectable_value=4, number_of_rows_sgadvanced=, number_of_rows=constant, number_of_columns_constant_value=15, col_port_width=4, minimum_columns=15, number_of_columns_selectable_value=4, number_of_columns_sgadvanced=, number_of_columns=constant, row_permutations_sgadvanced=, row_permutations=none, column_permutations_sgadvanced=, column_permutations=none, coe_file='no_coe_file_loaded', block_size_constant_value=225, block_size_port_width=8, block_size_type_sgadvanced=, block_size_type=rows_columns, has_aclken_sgadvanced=, has_aclken=off, has_aresetn_sgadvanced=, has_aresetn=off, infoeditControl=ARESETn must be asserted for a minmum of 2 cycles, has_col_valid_sgadvanced=, has_col_valid=off, has_col_sel_valid_sgadvanced=, has_col_sel_valid=off, has_row_valid_sgadvanced=, has_row_valid=off, has_row_sel_valid_sgadvanced=, has_row_sel_valid=off, has_block_size_valid_sgadvanced=, has_block_size_valid=off, has_dout_tready_sgadvanced=, has_dout_tready=off, has_fdo_sgadvanced=, has_fdo=off, has_rdy_sgadvanced=, has_rdy=off, has_block_start_sgadvanced=, has_block_start=off, has_block_end_sgadvanced=, has_block_end=off, pipelining_sgadvanced=, pipelining=maximum, trim_axipin_name=on, ip_name=Interleaver/De-interleaver, ip_version=7.0, dsptool_ready=true, ipcore_usecache=true, ipcore_useipmodelcache=true, wrapper_available=true, port_translation_map={ 'aclken' => 'en', 'aresetn' => 'rst'}, structural_sim=false, ipcore_verbose=false, ipcore_do_not_force_period=true, has_advanced_control=0, sggui_pos=-1,-1,-1,-1, block_type=sid_v7_0, block_version=, sg_icon_stat=215,202,3,5,white,green,0,457d4ab3,right,,[2 2 2 ],[2 3 3 3 1 ], sg_mask_display=|, sg_list_contents=, sg_blockgui_xml=}
      mask sg_mask_display=|
      | fprintf('','COMMENT: begin icon graphics');
      | patch([0 0 4 4 ],[188 14 14 188 ],[5.133333e-001 5.933333e-001 5.000000e-001 ]);
      | patch([211 211 215 215 ],[195 167 167 195 ],[5.133333e-001 5.933333e-001 5.000000e-001 ]);
      | patch([211 211 215 215 ],[155 47 47 155 ],[3.066667e-001 3.466667e-001 3.000000e-001 ]);
      | patch([211 211 215 215 ],[35 7 7 35 ],[7.200000e-001 8.400000e-001 7.000000e-001 ]);
      | patch([4 210 210 4 4 ],[0 0 202 202 0 ],[7.200000e-001 8.400000e-001 7.000000e-001 ]);
      | plot([4 210 210 4 4 ],[0 0 202 202 0 ]);
      |
      |
      | patch([44.7 85.16 113.16 141.16 169.16 113.16 72.7 44.7 ],[132.08 132.08 160.08 132.08 160.08 160.08 160.08 132.08 ],[1 1 1 ]);
      | patch([72.7 113.16 85.16 44.7 72.7 ],[104.08 104.08 132.08 132.08 104.08 ],[0.916 0.952 0.91 ]);
      | patch([44.7 85.16 113.16 72.7 44.7 ],[76.08 76.08 104.08 104.08 76.08 ],[1 1 1 ]);
      | patch([72.7 169.16 141.16 113.16 85.16 44.7 72.7 ],[48.08 48.08 76.08 48.08 76.08 76.08 48.08 ],[0.916 0.952 0.91 ]);
      | fprintf('','COMMENT: end icon graphics');
      | fprintf('','COMMENT: begin icon text');
      | color('black');port_label('input',1,'  data_tvalid  ');
      | color('black');port_label('input',2,'  data_tdata_din  ');
      | color('black');port_label('input',3,'  data_tlast  ');
      | color('black');port_label('output',1,'  data_tready  ');
      | color('black');port_label('output',2,'  data_tvalid  ');
      | color('black');port_label('output',3,'  data_tdata_dout  ');
      | color('black');port_label('output',4,'  data_tlast  ');
      | color('black');port_label('output',5,'  event_tlast_unexpected  ');
      | fprintf('','COMMENT: end icon text');
      mask prompts: infoedit ""; memory_style "Memory style"; symbol_width "Symbol Width"; sid_type_sgadvanced ""; sid_type ""; mode_sgadvanced ""; mode ""; external_memory_latency "External Symbol Memory Latency"; symbol_memory_sgadvanced ""; symbol_memory ""; number_of_branches "Number of branches"; architecture_sgadvanced ""; architecture ""; number_of_configurations "Number of configurations"; branch_length_type_sgadvanced ""; branch_length_type "Branch length descriptions for Forney SID"; branch_length_constant "Value"; branch_length_coe_file_name "COE File"; number_of_rows_constant_value "Value"; row_port_width "Row Port Width"; minimum_rows "Minimum Number of Rows"; number_of_rows_selectable_value "Number of Values"; number_of_rows_sgadvanced ""; number_of_rows ""; number_of_columns_constant_value "Value"; col_port_width "COL Port Width"; minimum_columns "Minimum Number of Columns"; number_of_columns_selectable_value "Number of Values"; number_of_columns_sgadvanced ""; number_of_columns ""; row_permutations_sgadvanced ""; row_permutations "Row Permutations"; column_permutations_sgadvanced ""; column_permutations "Column Permutations"; coe_file "COE File"; block_size_constant_value "Value"; block_size_port_width "BLOCK_SIZE Port Width"; block_size_type_sgadvanced ""; block_size_type ""; has_aclken_sgadvanced ""; has_aclken "ACLKEN"; has_aresetn_sgadvanced ""; has_aresetn "ARESETn (Active Low)."; infoeditControl ""; has_col_valid_sgadvanced ""; has_col_valid "COL_VALID"; has_col_sel_valid_sgadvanced ""; has_col_sel_valid "COL_SEL_VALID"; has_row_valid_sgadvanced ""; has_row_valid "ROW_VALID"; has_row_sel_valid_sgadvanced ""; has_row_sel_valid "ROW_SEL_VALID"; has_block_size_valid_sgadvanced ""; has_block_size_valid "BLOCK_SIZE_VALID"; has_dout_tready_sgadvanced ""; has_dout_tready "TREADY"; has_fdo_sgadvanced ""; has_fdo "FDO"; has_rdy_sgadvanced ""; has_rdy "RDY"; has_block_start_sgadvanced ""; has_block_start "BLOCK_START"; has_block_end_sgadvanced ""; has_block_end "BLOCK_END"; pipelining_sgadvanced ""; pipelining ""; trim_axipin_name "Display shortened port names"; ip_name ""; ip_version ""; dsptool_ready ""; ipcore_usecache ""; ipcore_useipmodelcache ""; wrapper_available ""; port_translation_map ""; structural_sim ""; ipcore_verbose ""; ipcore_do_not_force_period ""; has_advanced_control ""; sggui_pos ""; block_type ""; block_version ""; sg_icon_stat ""; sg_mask_display ""; sg_list_contents ""; sg_blockgui_xml ""
      mask help:
      | Forney Information : The Forney type is composed of a user-defined number of delay-line shift registers. The length of each of the delay-line shift registers can be specified using a COE file, or by setting the difference in the length of consecutive delay line shift registers to a fixed, user-defined value.
      |  Rectangular Information : The Rectangular Block type is composed of a rectangular array of memory elements, where the number of rows and columns in the array is user-defined. The number of rows and columns can be constant or run-time configurable. The elements are written to row-wise, and read out column-wise, or vice versa, depending on which mode is selected. This type supports user-defined inter-row and inter-column permutations. It also supports pruning - cases where the block size is less than the product of the number of rows and columns.
      mask init:
      | try
      |   tmp_gcb = gcb;
      |   tmp_gcbh = gcbh;
      |   if (strcmp('SysGenIndex',get_param(bdroot(tmp_gcbh),'tag')) && ~isempty(regexp(bdroot(tmp_gcb), '^xbs', 'once')))
      |     return;
      |   end;
      |   xlMungeMaskParams;
      |   block_config = 'sysgen:coregenimport_config';
      | 
      |   block_type='sid_v7_0';
      | 
      |   serialized_declarations = '{''architecture''=>''String'',''block_size_constant_value''=>''Int'',''block_size_port_width''=>''Int'',''block_size_type''=>''String'',''branch_length_coe_file_name''=>''String'',''branch_length_constant''=>''Int'',''branch_length_type''=>''String'',''coe_file''=>''String'',''col_port_width''=>''Int'',''column_permutations''=>''String'',''dsptool_ready''=>''Bool'',''external_memory_latency''=>''Int'',''has_aclken''=>''Bool'',''has_aresetn''=>''Bool'',''has_block_end''=>''Bool'',''has_block_size_valid''=>''Bool'',''has_block_start''=>''Bool'',''has_col_sel_valid''=>''Bool'',''has_col_valid''=>''Bool'',''has_dout_tready''=>''Bool'',''has_fdo''=>''Bool'',''has_rdy''=>''Bool'',''has_row_sel_valid''=>''Bool'',''has_row_valid''=>''Bool'',''ip_name''=>''String'',''ip_version''=>''String'',''ipcore_do_not_force_period''=>''Bool'',''ipcore_usecache''=>''Bool'',''ipcore_useipmodelcache''=>''Bool'',''ipcore_verbose''=>''Bool'',''memory_style''=>''String'',''minimum_columns''=>''Int'',''minimum_rows''=>''Int'',''mode''=>''String'',''number_of_branches''=>''Int'',''number_of_columns''=>''String'',''number_of_columns_constant_value''=>''Int'',''number_of_columns_selectable_value''=>''Int'',''number_of_configurations''=>''Int'',''number_of_rows''=>''String'',''number_of_rows_constant_value''=>''Int'',''number_of_rows_selectable_value''=>''Int'',''pipelining''=>''String'',''port_translation_map''=>''String'',''row_permutations''=>''String'',''row_port_width''=>''Int'',''sid_type''=>''String'',''structural_sim''=>''Bool'',''symbol_memory''=>''String'',''symbol_width''=>''Int'',''trim_axipin_name''=>''Int'',''wrapper_available''=>''Bool'',''block_type''=>''String''}';
      |   ptable_ = xlblockprep(get_param(tmp_gcb, 'MaskWSVariables'));
      |   try
      |     xlBlockMoveCallback(tmp_gcbh);
      |   catch 
      |      clear global xl_updateicon_recursion_guard;
      |   end;
      | catch
      |   global dbgsysgen;
      |   if(~isempty(dbgsysgen) && dbgsysgen)
      |     e = regexprep(lasterr, '\n', '\nError: ');
      |     disp(['Error: While running MaskInit code on block ' tmp_gcb ': ' e]);
      |     error(e);
      |   end
      | end
      settings: CopyFcn=xlBlockMoveCallback(gcbh);  DeleteFcn=xlDestroyGui(gcbh);  ModelCloseFcn=xlDestroyGui(gcbh);  PreSaveFcn=xlBlockPreSaveCallback(gcbh);  PostSaveFcn=xlBlockPostSaveCallback(gcbh);  DestroyFcn=xlDestroyGui(gcbh);  OpenFcn=xlOpenGui(gcbh, 'sid_v7_0_gui.xml', @sid_v6_0_enablement, @sid_v6_0_action)  CloseFcn=xlDestroyGui(gcbh);  MoveFcn=xlBlockMoveCallback(gcbh);
      mask Help: eval('');xlDoc('-book','sysgen','-topic','Interleaver__De_interleaver_7_0');
      mask StyleString: edit,popup(automatic|block|distributed),edit,edit,popup(forney|rectangular),edit,popup(interleaver|deinterleaver),edit,edit,popup(internal|external),edit,edit,popup(rom_based|logic_based),edit,edit,popup(constant_difference_between_consecutive_branches|use_coe_file_to_define_branch_lengths|coe_file_defines_branch_length_constant_for_each_configuration|coe_file_defines_individual_branch_lengths_for_every_branch_in_each_configuration),edit,edit,edit,edit,edit,edit,edit,popup(constant|variable|selectable),edit,edit,edit,edit,edit,popup(constant|variable|selectable),edit,popup(none|use_coe_file_to_define_row_permutations),edit,popup(none|use_coe_file_to_define_column_permutations),edit,edit,edit,edit,popup(constant|rows_columns|variable),edit,checkbox,edit,checkbox,edit,edit,checkbox,edit,checkbox,edit,checkbox,edit,checkbox,edit,checkbox,edit,checkbox,edit,checkbox,edit,checkbox,edit,checkbox,edit,checkbox,edit,popup(minimum|medium|maximum),checkbox,edit,edit,edit,edit,edit,edit,edit,edit,edit,edit,edit,edit,edit,edit,edit,edit,edit,edit
      mask Display:
      | fprintf('','COMMENT: begin icon graphics');
      | patch([0 0 4 4 ],[188 14 14 188 ],[5.133333e-001 5.933333e-001 5.000000e-001 ]);
      | patch([211 211 215 215 ],[195 167 167 195 ],[5.133333e-001 5.933333e-001 5.000000e-001 ]);
      | patch([211 211 215 215 ],[155 47 47 155 ],[3.066667e-001 3.466667e-001 3.000000e-001 ]);
      | patch([211 211 215 215 ],[35 7 7 35 ],[7.200000e-001 8.400000e-001 7.000000e-001 ]);
      | patch([4 210 210 4 4 ],[0 0 202 202 0 ],[7.200000e-001 8.400000e-001 7.000000e-001 ]);
      | plot([4 210 210 4 4 ],[0 0 202 202 0 ]);
      | 
      | 
      | patch([44.7 85.16 113.16 141.16 169.16 113.16 72.7 44.7 ],[132.08 132.08 160.08 132.08 160.08 160.08 160.08 132.08 ],[1 1 1 ]);
      | patch([72.7 113.16 85.16 44.7 72.7 ],[104.08 104.08 132.08 132.08 104.08 ],[0.916 0.952 0.91 ]);
      | patch([44.7 85.16 113.16 72.7 44.7 ],[76.08 76.08 104.08 104.08 76.08 ],[1 1 1 ]);
      | patch([72.7 169.16 141.16 113.16 85.16 44.7 72.7 ],[48.08 48.08 76.08 48.08 76.08 76.08 48.08 ],[0.916 0.952 0.91 ]);
      | fprintf('','COMMENT: end icon graphics');
      | fprintf('','COMMENT: begin icon text');
      | color('black');port_label('input',1,'  data_tvalid  ');
      | color('black');port_label('input',2,'  data_tdata_din  ');
      | color('black');port_label('input',3,'  data_tlast  ');
      | color('black');port_label('output',1,'  data_tready  ');
      | color('black');port_label('output',2,'  data_tvalid  ');
      | color('black');port_label('output',3,'  data_tdata_dout  ');
      | color('black');port_label('output',4,'  data_tlast  ');
      | color('black');port_label('output',5,'  event_tlast_unexpected  ');
      | fprintf('','COMMENT: end icon text');
  Inverter : S-Function  LoadFcn=xlBlockLoadCallback(gcbh);  FunctionName=sysgen  Parameters=ptable_  EnableBusSupport=off  mask(Xilinx Inverter Block){infoedit=Bitwise logical negation (one's complement) operator., en_sgadvanced=, en=off, latency=0, dbl_ovrd_sgadvanced=, dbl_ovrd=off, xl_use_area_sgadvanced=, xl_use_area=off, xl_area=[0,0,0,0,0,0,0], has_advanced_control=0, sggui_pos=-1,-1,-1,-1, block_type=inv, block_version=, sg_icon_stat=55,58,1,1,white,blue,0,267846e5,right,,[ ],[ ], sg_mask_display=|, sg_list_contents=, sg_blockgui_xml=}
      mask sg_mask_display=|
      | fprintf('','COMMENT: begin icon graphics');
      | patch([0 55 55 0 0 ],[0 0 58 58 0 ],[0.77 0.82 0.91 ]);
      | plot([0 55 55 0 0 ],[0 0 58 58 0 ]);
      | patch([11.425 21.54 28.54 35.54 42.54 28.54 18.425 11.425 ],[36.77 36.77 43.77 36.77 43.77 43.77 43.77 36.77 ],[1 1 1 ]);
      | patch([18.425 28.54 21.54 11.425 18.425 ],[29.77 29.77 36.77 36.77 29.77 ],[0.931 0.946 0.973 ]);
      | patch([11.425 21.54 28.54 18.425 11.425 ],[22.77 22.77 29.77 29.77 22.77 ],[1 1 1 ]);
      | patch([18.425 42.54 35.54 28.54 21.54 11.425 18.425 ],[15.77 15.77 22.77 15.77 22.77 22.77 15.77 ],[0.931 0.946 0.973 ]);
      | fprintf('','COMMENT: end icon graphics');
      | fprintf('','COMMENT: begin icon text');
      |
      |
      | color('black');disp('not');
      | fprintf('','COMMENT: end icon text');
      mask prompts: infoedit ""; en_sgadvanced ""; en "Provide enable port"; dbl_ovrd_sgadvanced ""; dbl_ovrd "Override with doubles"; xl_use_area_sgadvanced ""; xl_use_area "Define FPGA area for resource estimation"; xl_area "FPGA area [slices, FFs, BRAMs, LUTs, IOBs, emb. mults, TBUFs]"; has_advanced_control ""; sggui_pos ""; block_type ""; block_version ""; sg_icon_stat ""; sg_mask_display ""; sg_list_contents ""; sg_blockgui_xml ""
      mask help: Bitwise logical negation (one's complement) operator.
      mask init:
      | try
      |   tmp_gcb = gcb;
      |   tmp_gcbh = gcbh;
      |   if (strcmp('SysGenIndex',get_param(bdroot(tmp_gcbh),'tag')) && ~isempty(regexp(bdroot(tmp_gcb), '^xbs', 'once')))
      |     return;
      |   end;
      |   xlMungeMaskParams;
      |   block_config = 'sysgen_blockset:Inverter_config';
      | 
      |   block_type='inv';
      | 
      |   serialized_declarations = '{''dbl_ovrd''=>''Int'',''en''=>''Int'',''latency''=>''Int'',''block_type''=>''String''}';
      |   ptable_ = xlblockprep(get_param(tmp_gcb, 'MaskWSVariables'));
      |   try
      |     xlBlockMoveCallback(tmp_gcbh);
      |   catch 
      |      clear global xl_updateicon_recursion_guard;
      |   end;
      | catch
      |   global dbgsysgen;
      |   if(~isempty(dbgsysgen) && dbgsysgen)
      |     e = regexprep(lasterr, '\n', '\nError: ');
      |     disp(['Error: While running MaskInit code on block ' tmp_gcb ': ' e]);
      |     error(e);
      |   end
      | end
      settings: CopyFcn=xlBlockMoveCallback(gcbh);  DeleteFcn=xlDestroyGui(gcbh);  ModelCloseFcn=xlDestroyGui(gcbh);  PreSaveFcn=xlBlockPreSaveCallback(gcbh);  PostSaveFcn=xlBlockPostSaveCallback(gcbh);  DestroyFcn=xlDestroyGui(gcbh);  OpenFcn=xlOpenGui(gcbh, 'inv_gui.xml', @xlmagicenablement, -1)  CloseFcn=xlDestroyGui(gcbh);  MoveFcn=xlBlockMoveCallback(gcbh);
      mask Help: eval('');xlDoc('-book','sysgen','-topic','Inverter');
      mask Display:
      | fprintf('','COMMENT: begin icon graphics');
      | patch([0 55 55 0 0 ],[0 0 58 58 0 ],[0.77 0.82 0.91 ]);
      | plot([0 55 55 0 0 ],[0 0 58 58 0 ]);
      | patch([11.425 21.54 28.54 35.54 42.54 28.54 18.425 11.425 ],[36.77 36.77 43.77 36.77 43.77 43.77 43.77 36.77 ],[1 1 1 ]);
      | patch([18.425 28.54 21.54 11.425 18.425 ],[29.77 29.77 36.77 36.77 29.77 ],[0.931 0.946 0.973 ]);
      | patch([11.425 21.54 28.54 18.425 11.425 ],[22.77 22.77 29.77 29.77 22.77 ],[1 1 1 ]);
      | patch([18.425 42.54 35.54 28.54 21.54 11.425 18.425 ],[15.77 15.77 22.77 15.77 22.77 22.77 15.77 ],[0.931 0.946 0.973 ]);
      | fprintf('','COMMENT: end icon graphics');
      | fprintf('','COMMENT: begin icon text');
      | 
      | 
      | color('black');disp('not');
      | fprintf('','COMMENT: end icon text');
  LFSR : S-Function  LoadFcn=xlBlockLoadCallback(gcbh);  FunctionName=sysgen  Parameters=ptable_  EnableBusSupport=off  mask(Xilinx Linear Feedback Shift Register Block){lfsr_type_sgadvanced=, lfsr_type=Fibonacci, gate_type_sgadvanced=, gate_type=XOR, n_bits=6, polynomial='11', rst_value='3F', rst_sgadvanced=, rst=off, en_sgadvanced=, en=off, reloadable_seed_sgadvanced=, reloadable_seed=off, input_type_sgadvanced=, input_type=off, output_type_sgadvanced=, output_type=off, arith_type_sgadvanced=, arith_type=Signed  (2's comp), bin_pt=4, dbl_ovrd_sgadvanced=, dbl_ovrd=off, explicit_period_sgadvanced=, explicit_period=off, period=1, xl_use_area_sgadvanced=, xl_use_area=off, xl_area=[0,0,0,0,0,0,0], has_advanced_control=0, sggui_pos=-1,-1,-1,-1, block_type=lfsr, block_version=, sg_icon_stat=60,60,0,1,white,blue,0,b27a07ff,right,,[ ],[ ], sg_mask_display=|, sg_list_contents=, sg_blockgui_xml=}
      mask sg_mask_display=|
      | fprintf('','COMMENT: begin icon graphics');
      | patch([0 60 60 0 0 ],[0 0 60 60 0 ],[0.77 0.82 0.91 ]);
      | plot([0 60 60 0 0 ],[0 0 60 60 0 ]);
      | patch([12.2 23.76 31.76 39.76 47.76 31.76 20.2 12.2 ],[38.88 38.88 46.88 38.88 46.88 46.88 46.88 38.88 ],[1 1 1 ]);
      | patch([20.2 31.76 23.76 12.2 20.2 ],[30.88 30.88 38.88 38.88 30.88 ],[0.931 0.946 0.973 ]);
      | patch([12.2 23.76 31.76 20.2 12.2 ],[22.88 22.88 30.88 30.88 22.88 ],[1 1 1 ]);
      | patch([20.2 47.76 39.76 31.76 23.76 12.2 20.2 ],[14.88 14.88 22.88 14.88 22.88 22.88 14.88 ],[0.931 0.946 0.973 ]);
      | fprintf('','COMMENT: end icon graphics');
      | fprintf('','COMMENT: begin icon text');
      | color('black');port_label('output',1,'dout');
      | fprintf('','COMMENT: end icon text');
      mask prompts: lfsr_type_sgadvanced ""; lfsr_type "Type"; gate_type_sgadvanced ""; gate_type "Gate type"; n_bits "Number of bits in LFSR"; polynomial "Feedback polynomial (enter hex value enclosed with ticks)"; rst_value "Initial value (enter hex value enclosed with ticks)"; rst_sgadvanced ""; rst "Provide synchronous reset port"; en_sgadvanced ""; en "Provide enable port"; reloadable_seed_sgadvanced ""; reloadable_seed "Use reloadable seed values"; input_type_sgadvanced ""; input_type "Parallel input"; output_type_sgadvanced ""; output_type "Parallel output"; arith_type_sgadvanced ""; arith_type "Output type"; bin_pt "Binary point"; dbl_ovrd_sgadvanced ""; dbl_ovrd "Override with doubles"; explicit_period_sgadvanced ""; explicit_period "Specify explicit sample period"; period ""; xl_use_area_sgadvanced ""; xl_use_area "Define FPGA area for resource estimation"; xl_area "FPGA area [slices, FFs, BRAMs, LUTs, IOBs, emb. mults, TBUFs]"; has_advanced_control ""; sggui_pos ""; block_type ""; block_version ""; sg_icon_stat ""; sg_mask_display ""; sg_list_contents ""; sg_blockgui_xml ""
      mask help: Xilinx Linear Feedback Shift Register
      mask init:
      | try
      |   tmp_gcb = gcb;
      |   tmp_gcbh = gcbh;
      |   if (strcmp('SysGenIndex',get_param(bdroot(tmp_gcbh),'tag')) && ~isempty(regexp(bdroot(tmp_gcb), '^xbs', 'once')))
      |     return;
      |   end;
      |   xlMungeMaskParams;
      |   block_config = 'sysgen_blockset:LFSR_config';
      | 
      |   block_type='lfsr';
      | 
      |   serialized_declarations = '{''arith_type''=>''Int'',''bin_pt''=>''Int'',''dbl_ovrd''=>''Int'',''en''=>''Int'',''explicit_period''=>''Int'',''gate_type''=>''Int'',''infoedit''=>''String'',''init''=>''String'',''input_type''=>''Int'',''lfsr_type''=>''Int'',''n_bits''=>''Int'',''output_type''=>''Int'',''period''=>''Double'',''polynomial''=>''String'',''reloadable_seed''=>''Int'',''rst''=>''Int'',''rst_vale''=>''String'',''rst_value''=>''String'',''sim_engine''=>''Int'',''sysgen_root''=>''String'',''xl_use_area''=>''Int'',''block_type''=>''String''}';
      |   xllfsr_init();
      |   ptable_ = xlblockprep(get_param(tmp_gcb, 'MaskWSVariables'));
      |   try
      |     xlBlockMoveCallback(tmp_gcbh);
      |   catch 
      |      clear global xl_updateicon_recursion_guard;
      |   end;
      | catch
      |   global dbgsysgen;
      |   if(~isempty(dbgsysgen) && dbgsysgen)
      |     e = regexprep(lasterr, '\n', '\nError: ');
      |     disp(['Error: While running MaskInit code on block ' tmp_gcb ': ' e]);
      |     error(e);
      |   end
      | end
